simulink model "Der_Faux_FPGA_V2_optimized_synthesizable"  (R2020a)
settings: Solver=FixedStepDiscrete  StartTime=0.0  StopTime=0.84375  FixedStep=1/fs_sim  RelTol=1e-3
values from neighbouring files (symbols this model uses):
  ADC_res = 5    [Der_Faux_ctr_FPGA.m]
  ADC_res_G4 = 8    [Der_Faux_ctr_FPGA.m]
  fs = 48000    [Der_Faux_ctr_FPGA.m]
  fs_sim = fs*ovs    (= 6144000)    [Der_Faux_ctr_FPGA.m]
  Gvar1_N = fi(Gvar1_N,0,ADC_res,0)    [Der_Faux_ctr_FPGA.m]
  Gvar2_N = fi(Gvar2_N,0,ADC_res,0)    [Der_Faux_ctr_FPGA.m]
  Gvar3_N = fi(Gvar3_N,0,ADC_res,0)    [Der_Faux_ctr_FPGA.m]
  Gvar4_N = fi(Gvar4_N,0,ADC_res_G4,0)    [Der_Faux_ctr_FPGA.m]
  input_space = linspace(0,2^ADC_res-1,2^ADC_res)    [Der_Faux_ctr_FPGA.m]
  input_spcae_extended = linspace(0,(2^ADC_res)^3-1,(2^ADC_res)^3)    [Der_Faux_ctr_FPGA.m]
  LUT_Z22a_opt = sfi(LUT_Z22a, len_LUT22a)    [Der_Faux_ctr_FPGA.m]
  LUT_Z22b_opt = sfi(LUT_Z22b, len_LUT22b)    [Der_Faux_ctr_FPGA.m]
  LUT_Z23a_opt = sfi(LUT_Z23a, len_Z23a)    [Der_Faux_ctr_FPGA.m]
  LUT_Z23b_opt = sfi(LUT_Z23b, len_Z23b)    [Der_Faux_ctr_FPGA.m]
  LUT_Z24a_opt = sfi(LUT_Z24a, len_LUT24a)    [Der_Faux_ctr_FPGA.m]
  LUT_Z24b_opt = sfi(LUT_Z24b, len_LUT24b)    [Der_Faux_ctr_FPGA.m]
  LUT_Z25a_opt = sfi(LUT_Z25a, len_LUT25a)    [Der_Faux_ctr_FPGA.m]
  LUT_Z25b_opt = sfi(LUT_Z25b, len_LUT25b)    [Der_Faux_ctr_FPGA.m]
  shift_reg_size = 8*44000    (= 352000)    [Der_Faux_ctr_FPGA.m]
  use_stimuli = [true,true,true,true]    [Der_Faux_ctr_FPGA.m]
  WL_RAM = 5    [Der_Faux_ctr_FPGA.m]
undefined symbols (not defined in the file or in its folder): poti_stimuli1, poti_stimuli2, poti_stimuli3, poti_stimuli4
libraries: hdlmdlgenlib x30, simulink x6, hdlsllib x4
(part 2 of 3)

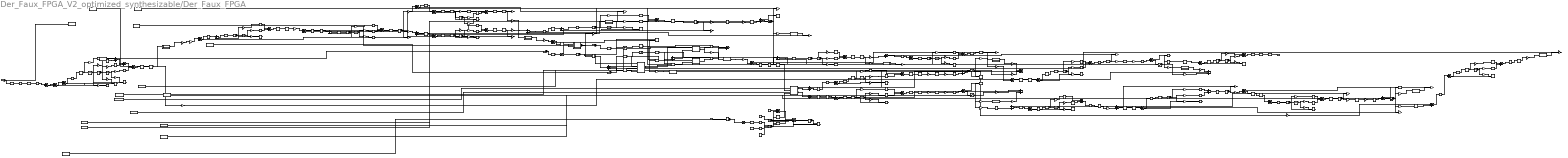
== system Der_Faux_FPGA_V2_optimized_synthesizable/Der_Faux_FPGA ==
  Vin : Inport  OutDataTypeStr=fixdt(1, 16, 15)  PortDimensions=1  SampleTime=2.08333333333333e-05  LockScale=on
  Gvar1_N : Inport  Port=2  OutDataTypeStr=fixdt(0, 5, 0)  PortDimensions=1  SampleTime=1.62760416666667e-07  LockScale=on
  Gvar2_N : Inport  Port=3  OutDataTypeStr=fixdt(0, 5, 0)  PortDimensions=1  SampleTime=1.62760416666667e-07  LockScale=on
  Gvar3_N : Inport  Port=4  OutDataTypeStr=fixdt(0, 5, 0)  PortDimensions=1  SampleTime=1.62760416666667e-07  LockScale=on
  Gvar4_N : Inport  Port=5  OutDataTypeStr=uint8  PortDimensions=1  SampleTime=1.62760416666667e-07  LockScale=on
  1-D Lookup Table1 : Lookup_n-D  NumberOfTableDimensions=1  BreakpointsForDimension1="fi(\"numerictype\",numerictype(0,8,0),\"fimath\",fimath(\"RoundingMethod\", \"Nearest\",\"OverflowAction\", \"Saturate\",\"ProductMode\",\"FullPrecision\",\"SumMode\",\"FullPrecision\"),\"Value\",\"[0 1 2 3 4 5 6 7 8 9 10 11 12 13 14 15 16 17 18 19 20 21 22 23 24 25 26 27 28 29 30 31 32 33 34 35 36 37 38 39 40 41 42 43 44 45 46 47 48 49 50 51 52 53 54 55 56 57 58 59 60 61 62 63 64 65 66 67 68 69 70 71 72 73 74 75 76 77 78 79 80 81 82 83 84 85 86 87 88 89 90 91 92 93 94 95 96 97 98 99 100 101 102 103 104 105 106 107 108 109 110 111 112 113 114 115 116 117 118 119 120 121 122 123 124 125 126 127 128 129 130 131 132 133 134 135 136 137 138 139 140 141 142 143 144 145 146 147 148 149 150 151 152 153 154 155 156 157 158 159 160 161 162 163 164 165 166 167 168 169 170 171 172 173 174 175 176 177 178 179 180 181 182 183 184 185 186 187 188 189 190 191 192 193 194 195 196 197 198 199 200 201 202 203 204 205 206 207 208 209 210 211 212 213 214 215 216 217 218 219 220 221 222 223 224 225 226 227 228 229 230 231 232 233 234 235 236 237 238 239 240 241 242 243 244 245 246 247 248 249 250 251 252 253 254 255]\")"  Table="reshape(fi(\"numerictype\",numerictype(0,4,0),\"fimath\",fimath(\"RoundingMethod\", \"Floor\",\"OverflowAction\", \"Wrap\",\"ProductMode\",\"FullPrecision\",\"SumMode\",\"FullPrecision\"),\"Value\",\"[1;1;1;1;1;1;1;1;1;1;1;1;1;1;1;1;1;1;1;1;1;1;1;1;1;1;1;1;1;1;1;1;1;1;1;1;1;1;1;1;1;1;1;1;1;1;1;1;1;1;1;2;2;2;2;2;2;2;2;2;2;2;2;2;2;2;2;2;2;2;2;2;2;2;2;2;3;3;3;3;3;3;3;3;3;3;3;3;3;3;3;3;3;3;3;3;3;3;3;3;3;3;4;4;4;4;4;4;4;4;4;4;4;4;4;4;4;4;4;4;4;4;4;4;4;4;4;5;5;5;5;5;5;5;5;5;5;5;5;5;5;5;5;5;5;5;5;5;5;5;5;5;5;6;6;6;6;6;6;6;6;6;6;6;6;6;6;6;6;6;6;6;6;6;6;6;6;6;7;7;7;7;7;7;7;7;7;7;7;7;7;7;7;7;7;7;7;7;7;7;7;7;7;7;8;8;8;8;8;8;8;8;8;8;8;8;8;8;8;8;8;8;8;8;8;8;8;8;8;9;9;9;9;9;9;9;9;9;9;9;9;9;9;9;9;9;9;9;9;9;9;9;9;9;9;10]\"), [1  256])"  InterpMethod=Flat  ExtrapMethod=Clip  DiagnosticForOutOfRangeInput=Error  SampleTime=1.62760416666667e-07  OutDataTypeStr=fixdt(0, 4, 0)  RndMeth=Simplest  InputSameDT=on
  Comparator Logic : Subsystem
  Compare To Zero2 : simulink/Logic and Bit Operations/Compare To Constant  relop===  const=double(0)  OutDataTypeStr=boolean
  Constant14 : Constant  Value=0  OutDataTypeStr=fixdt(0, 4, 0)  SampleTime=1.62760416666667e-07
  Constant8 : Constant  OutDataTypeStr=fixdt(0, 4, 0)  SampleTime=1.62760416666667e-07
  Data Type Conversion : DataTypeConversion  OutDataTypeStr=fixdt(1, 46, 44)  SampleTime=2.08333333333333e-05  SaturateOnIntegerOverflow=on
  Data Type Conversion1 : DataTypeConversion  OutDataTypeStr=fixdt(1, 16, 15)  SampleTime=2.08333333333333e-05  SaturateOnIntegerOverflow=on
  Data Type Conversion2 : DataTypeConversion  OutDataTypeStr=fixdt(0, 4, 0)  SampleTime=1.62760416666667e-07
  Delay Mod{1..6,8..9} (8 alike) : Delay  DelayLength=double(1)  InitialCondition=0  SampleTime=1.62760416666667e-07
  Delay1 : Delay  DelayLength=double(1)  InitialCondition=0  SampleTime=1.62760416666667e-07
  Delay2 : Delay  DelayLength=double(1)  InitialCondition=0  SampleTime=1.62760416666667e-07
  Delay3 : Delay  DelayLength=double(1)  InitialCondition=0  SampleTime=1.62760416666667e-07
  Difference1 : Subsystem  mask(Difference){ICPrevInput=double(0), InputProcessing=Elements as channels (sample based), OutMin=[], OutMax=[], OutDataTypeStr=fixdt(1,46,81), OutputDataTypeScalingMode=Specify via dialog, OutDataType=fixdt(1,46,81), OutScaling=[], LockScale=off, RndMeth=Floor, DoSatur=on}
      mask prompts: ICPrevInput "Simulink:masks:InitialConditionForPreviousInput_MP"; InputProcessing "Simulink:masks:InputProcessing_MP"; OutMin "Simulink:masks:OutputMinimum_MP"; OutMax "Simulink:masks:OutputMaximum_MP"; OutDataTypeStr "Simulink:masks:OutputDataType_MP"; OutputDataTypeScalingMode "Simulink:masks:OutputDataTypeMode_MP"; OutDataType "Simulink:masks:OutputDataTypeegFixdt116Fixdtsingle_MP"; OutScaling "Simulink:masks:OutputScalingSlopeEg29OrSlopeBias_MP"; LockScale "Simulink:masks:LockOutputDataTypeAgainstFxpTools_MP"; RndMeth "Simulink:masks:IntegerRoundingMode_MP"; DoSatur "Simulink:masks:SaturateToMaxOrMinWhenOverflowsOccur_MP"
      mask help: Simulink:masks:Difference_MD
      mask init:
      | blkH = gcbh;
      | blkName = getfullname(blkH);
      | 
      | set_param([blkName,'/Diff'], ...
      |     'RndMeth',RndMeth, ...
      | 	'DoSatur',DoSatur);
      | 
      | set_param([blkName,'/UD'], ...
      | 	'InputProcessing',InputProcessing);
      mask TypeOptions InputProcessing: Simulink:masks:ColumnsAsChannelsFrameBased | Simulink:masks:ElementsAsChannelsSampleBased
      mask Callback OutDataTypeStr: fixptdialog(gcbh)
      mask TypeOptions OutputDataTypeScalingMode: double | single | int8 | uint8 | int16 | uint16 | int32 | uint32 | Specify via dialog | Inherit via internal rule | Inherit via back propagation
      mask Callback OutputDataTypeScalingMode: fixptdialog(gcbh)
      mask Callback OutDataType: fixptdialog(gcbh)
      mask TypeOptions RndMeth: Simulink:masks:Ceiling | Simulink:masks:Convergent | Simulink:masks:Floor | Simulink:masks:Nearest | Simulink:masks:Round | Simulink:masks:Simplest | Simulink:masks:Zero
      mask Display: dpoly([1 -1],[1 0],'z')
  Difference10 : Subsystem  mask(Difference){ICPrevInput=double(0), InputProcessing=Elements as channels (sample based), OutMin=[], OutMax=[], OutDataTypeStr=fixdt(1,46,77), OutputDataTypeScalingMode=Specify via dialog, OutDataType=fixdt(1,46,77), OutScaling=[], LockScale=off, RndMeth=Floor, DoSatur=on}
      mask prompts: ICPrevInput "Simulink:masks:InitialConditionForPreviousInput_MP"; InputProcessing "Simulink:masks:InputProcessing_MP"; OutMin "Simulink:masks:OutputMinimum_MP"; OutMax "Simulink:masks:OutputMaximum_MP"; OutDataTypeStr "Simulink:masks:OutputDataType_MP"; OutputDataTypeScalingMode "Simulink:masks:OutputDataTypeMode_MP"; OutDataType "Simulink:masks:OutputDataTypeegFixdt116Fixdtsingle_MP"; OutScaling "Simulink:masks:OutputScalingSlopeEg29OrSlopeBias_MP"; LockScale "Simulink:masks:LockOutputDataTypeAgainstFxpTools_MP"; RndMeth "Simulink:masks:IntegerRoundingMode_MP"; DoSatur "Simulink:masks:SaturateToMaxOrMinWhenOverflowsOccur_MP"
      mask help: Simulink:masks:Difference_MD
      mask init:
      | blkH = gcbh;
      | blkName = getfullname(blkH);
      | 
      | set_param([blkName,'/Diff'], ...
      |     'RndMeth',RndMeth, ...
      | 	'DoSatur',DoSatur);
      | 
      | set_param([blkName,'/UD'], ...
      | 	'InputProcessing',InputProcessing);
      mask TypeOptions InputProcessing: Simulink:masks:ColumnsAsChannelsFrameBased | Simulink:masks:ElementsAsChannelsSampleBased
      mask Callback OutDataTypeStr: fixptdialog(gcbh)
      mask TypeOptions OutputDataTypeScalingMode: double | single | int8 | uint8 | int16 | uint16 | int32 | uint32 | Specify via dialog | Inherit via internal rule | Inherit via back propagation
      mask Callback OutputDataTypeScalingMode: fixptdialog(gcbh)
      mask Callback OutDataType: fixptdialog(gcbh)
      mask TypeOptions RndMeth: Simulink:masks:Ceiling | Simulink:masks:Convergent | Simulink:masks:Floor | Simulink:masks:Nearest | Simulink:masks:Round | Simulink:masks:Simplest | Simulink:masks:Zero
      mask Display: dpoly([1 -1],[1 0],'z')
  Difference11 : Subsystem  mask(Difference){ICPrevInput=double(0), InputProcessing=Elements as channels (sample based), OutMin=[], OutMax=[], OutDataTypeStr=fixdt(1,46,77), OutputDataTypeScalingMode=Specify via dialog, OutDataType=fixdt(1,46,77), OutScaling=[], LockScale=off, RndMeth=Floor, DoSatur=on}
      mask prompts: ICPrevInput "Simulink:masks:InitialConditionForPreviousInput_MP"; InputProcessing "Simulink:masks:InputProcessing_MP"; OutMin "Simulink:masks:OutputMinimum_MP"; OutMax "Simulink:masks:OutputMaximum_MP"; OutDataTypeStr "Simulink:masks:OutputDataType_MP"; OutputDataTypeScalingMode "Simulink:masks:OutputDataTypeMode_MP"; OutDataType "Simulink:masks:OutputDataTypeegFixdt116Fixdtsingle_MP"; OutScaling "Simulink:masks:OutputScalingSlopeEg29OrSlopeBias_MP"; LockScale "Simulink:masks:LockOutputDataTypeAgainstFxpTools_MP"; RndMeth "Simulink:masks:IntegerRoundingMode_MP"; DoSatur "Simulink:masks:SaturateToMaxOrMinWhenOverflowsOccur_MP"
      mask help: Simulink:masks:Difference_MD
      mask init:
      | blkH = gcbh;
      | blkName = getfullname(blkH);
      | 
      | set_param([blkName,'/Diff'], ...
      |     'RndMeth',RndMeth, ...
      | 	'DoSatur',DoSatur);
      | 
      | set_param([blkName,'/UD'], ...
      | 	'InputProcessing',InputProcessing);
      mask TypeOptions InputProcessing: Simulink:masks:ColumnsAsChannelsFrameBased | Simulink:masks:ElementsAsChannelsSampleBased
      mask Callback OutDataTypeStr: fixptdialog(gcbh)
      mask TypeOptions OutputDataTypeScalingMode: double | single | int8 | uint8 | int16 | uint16 | int32 | uint32 | Specify via dialog | Inherit via internal rule | Inherit via back propagation
      mask Callback OutputDataTypeScalingMode: fixptdialog(gcbh)
      mask Callback OutDataType: fixptdialog(gcbh)
      mask TypeOptions RndMeth: Simulink:masks:Ceiling | Simulink:masks:Convergent | Simulink:masks:Floor | Simulink:masks:Nearest | Simulink:masks:Round | Simulink:masks:Simplest | Simulink:masks:Zero
      mask Display: dpoly([1 -1],[1 0],'z')
  Difference12 : Subsystem  mask(Difference){ICPrevInput=double(0), InputProcessing=Elements as channels (sample based), OutMin=[], OutMax=[], OutDataTypeStr=fixdt(1,46,73), OutputDataTypeScalingMode=Specify via dialog, OutDataType=fixdt(1,46,73), OutScaling=[], LockScale=off, RndMeth=Floor, DoSatur=on}
      mask prompts: ICPrevInput "Simulink:masks:InitialConditionForPreviousInput_MP"; InputProcessing "Simulink:masks:InputProcessing_MP"; OutMin "Simulink:masks:OutputMinimum_MP"; OutMax "Simulink:masks:OutputMaximum_MP"; OutDataTypeStr "Simulink:masks:OutputDataType_MP"; OutputDataTypeScalingMode "Simulink:masks:OutputDataTypeMode_MP"; OutDataType "Simulink:masks:OutputDataTypeegFixdt116Fixdtsingle_MP"; OutScaling "Simulink:masks:OutputScalingSlopeEg29OrSlopeBias_MP"; LockScale "Simulink:masks:LockOutputDataTypeAgainstFxpTools_MP"; RndMeth "Simulink:masks:IntegerRoundingMode_MP"; DoSatur "Simulink:masks:SaturateToMaxOrMinWhenOverflowsOccur_MP"
      mask help: Simulink:masks:Difference_MD
      mask init:
      | blkH = gcbh;
      | blkName = getfullname(blkH);
      | 
      | set_param([blkName,'/Diff'], ...
      |     'RndMeth',RndMeth, ...
      | 	'DoSatur',DoSatur);
      | 
      | set_param([blkName,'/UD'], ...
      | 	'InputProcessing',InputProcessing);
      mask TypeOptions InputProcessing: Simulink:masks:ColumnsAsChannelsFrameBased | Simulink:masks:ElementsAsChannelsSampleBased
      mask Callback OutDataTypeStr: fixptdialog(gcbh)
      mask TypeOptions OutputDataTypeScalingMode: double | single | int8 | uint8 | int16 | uint16 | int32 | uint32 | Specify via dialog | Inherit via internal rule | Inherit via back propagation
      mask Callback OutputDataTypeScalingMode: fixptdialog(gcbh)
      mask Callback OutDataType: fixptdialog(gcbh)
      mask TypeOptions RndMeth: Simulink:masks:Ceiling | Simulink:masks:Convergent | Simulink:masks:Floor | Simulink:masks:Nearest | Simulink:masks:Round | Simulink:masks:Simplest | Simulink:masks:Zero
      mask Display: dpoly([1 -1],[1 0],'z')
  Difference13 : Subsystem  mask(Difference){ICPrevInput=double(0), InputProcessing=Elements as channels (sample based), OutMin=[], OutMax=[], OutDataTypeStr=fixdt(1,46,73), OutputDataTypeScalingMode=Specify via dialog, OutDataType=fixdt(1,46,73), OutScaling=[], LockScale=off, RndMeth=Floor, DoSatur=on}
      mask prompts: ICPrevInput "Simulink:masks:InitialConditionForPreviousInput_MP"; InputProcessing "Simulink:masks:InputProcessing_MP"; OutMin "Simulink:masks:OutputMinimum_MP"; OutMax "Simulink:masks:OutputMaximum_MP"; OutDataTypeStr "Simulink:masks:OutputDataType_MP"; OutputDataTypeScalingMode "Simulink:masks:OutputDataTypeMode_MP"; OutDataType "Simulink:masks:OutputDataTypeegFixdt116Fixdtsingle_MP"; OutScaling "Simulink:masks:OutputScalingSlopeEg29OrSlopeBias_MP"; LockScale "Simulink:masks:LockOutputDataTypeAgainstFxpTools_MP"; RndMeth "Simulink:masks:IntegerRoundingMode_MP"; DoSatur "Simulink:masks:SaturateToMaxOrMinWhenOverflowsOccur_MP"
      mask help: Simulink:masks:Difference_MD
      mask init:
      | blkH = gcbh;
      | blkName = getfullname(blkH);
      | 
      | set_param([blkName,'/Diff'], ...
      |     'RndMeth',RndMeth, ...
      | 	'DoSatur',DoSatur);
      | 
      | set_param([blkName,'/UD'], ...
      | 	'InputProcessing',InputProcessing);
      mask TypeOptions InputProcessing: Simulink:masks:ColumnsAsChannelsFrameBased | Simulink:masks:ElementsAsChannelsSampleBased
      mask Callback OutDataTypeStr: fixptdialog(gcbh)
      mask TypeOptions OutputDataTypeScalingMode: double | single | int8 | uint8 | int16 | uint16 | int32 | uint32 | Specify via dialog | Inherit via internal rule | Inherit via back propagation
      mask Callback OutputDataTypeScalingMode: fixptdialog(gcbh)
      mask Callback OutDataType: fixptdialog(gcbh)
      mask TypeOptions RndMeth: Simulink:masks:Ceiling | Simulink:masks:Convergent | Simulink:masks:Floor | Simulink:masks:Nearest | Simulink:masks:Round | Simulink:masks:Simplest | Simulink:masks:Zero
      mask Display: dpoly([1 -1],[1 0],'z')
  Difference3 : Subsystem  mask(Difference){ICPrevInput=double(0), InputProcessing=Elements as channels (sample based), OutMin=[], OutMax=[], OutDataTypeStr=fixdt(1,46,47), OutputDataTypeScalingMode=Specify via dialog, OutDataType=fixdt(1,46,47), OutScaling=[], LockScale=off, RndMeth=Floor, DoSatur=on}
      mask prompts: ICPrevInput "Simulink:masks:InitialConditionForPreviousInput_MP"; InputProcessing "Simulink:masks:InputProcessing_MP"; OutMin "Simulink:masks:OutputMinimum_MP"; OutMax "Simulink:masks:OutputMaximum_MP"; OutDataTypeStr "Simulink:masks:OutputDataType_MP"; OutputDataTypeScalingMode "Simulink:masks:OutputDataTypeMode_MP"; OutDataType "Simulink:masks:OutputDataTypeegFixdt116Fixdtsingle_MP"; OutScaling "Simulink:masks:OutputScalingSlopeEg29OrSlopeBias_MP"; LockScale "Simulink:masks:LockOutputDataTypeAgainstFxpTools_MP"; RndMeth "Simulink:masks:IntegerRoundingMode_MP"; DoSatur "Simulink:masks:SaturateToMaxOrMinWhenOverflowsOccur_MP"
      mask help: Simulink:masks:Difference_MD
      mask init:
      | blkH = gcbh;
      | blkName = getfullname(blkH);
      | 
      | set_param([blkName,'/Diff'], ...
      |     'RndMeth',RndMeth, ...
      | 	'DoSatur',DoSatur);
      | 
      | set_param([blkName,'/UD'], ...
      | 	'InputProcessing',InputProcessing);
      mask TypeOptions InputProcessing: Simulink:masks:ColumnsAsChannelsFrameBased | Simulink:masks:ElementsAsChannelsSampleBased
      mask Callback OutDataTypeStr: fixptdialog(gcbh)
      mask TypeOptions OutputDataTypeScalingMode: double | single | int8 | uint8 | int16 | uint16 | int32 | uint32 | Specify via dialog | Inherit via internal rule | Inherit via back propagation
      mask Callback OutputDataTypeScalingMode: fixptdialog(gcbh)
      mask Callback OutDataType: fixptdialog(gcbh)
      mask TypeOptions RndMeth: Simulink:masks:Ceiling | Simulink:masks:Convergent | Simulink:masks:Floor | Simulink:masks:Nearest | Simulink:masks:Round | Simulink:masks:Simplest | Simulink:masks:Zero
      mask Display: dpoly([1 -1],[1 0],'z')
  Difference4 : Subsystem  mask(Difference){ICPrevInput=double(0), InputProcessing=Elements as channels (sample based), OutMin=[], OutMax=[], OutDataTypeStr=fixdt(1,46,82), OutputDataTypeScalingMode=Specify via dialog, OutDataType=fixdt(1,46,82), OutScaling=[], LockScale=off, RndMeth=Floor, DoSatur=on}
      mask prompts: ICPrevInput "Simulink:masks:InitialConditionForPreviousInput_MP"; InputProcessing "Simulink:masks:InputProcessing_MP"; OutMin "Simulink:masks:OutputMinimum_MP"; OutMax "Simulink:masks:OutputMaximum_MP"; OutDataTypeStr "Simulink:masks:OutputDataType_MP"; OutputDataTypeScalingMode "Simulink:masks:OutputDataTypeMode_MP"; OutDataType "Simulink:masks:OutputDataTypeegFixdt116Fixdtsingle_MP"; OutScaling "Simulink:masks:OutputScalingSlopeEg29OrSlopeBias_MP"; LockScale "Simulink:masks:LockOutputDataTypeAgainstFxpTools_MP"; RndMeth "Simulink:masks:IntegerRoundingMode_MP"; DoSatur "Simulink:masks:SaturateToMaxOrMinWhenOverflowsOccur_MP"
      mask help: Simulink:masks:Difference_MD
      mask init:
      | blkH = gcbh;
      | blkName = getfullname(blkH);
      | 
      | set_param([blkName,'/Diff'], ...
      |     'RndMeth',RndMeth, ...
      | 	'DoSatur',DoSatur);
      | 
      | set_param([blkName,'/UD'], ...
      | 	'InputProcessing',InputProcessing);
      mask TypeOptions InputProcessing: Simulink:masks:ColumnsAsChannelsFrameBased | Simulink:masks:ElementsAsChannelsSampleBased
      mask Callback OutDataTypeStr: fixptdialog(gcbh)
      mask TypeOptions OutputDataTypeScalingMode: double | single | int8 | uint8 | int16 | uint16 | int32 | uint32 | Specify via dialog | Inherit via internal rule | Inherit via back propagation
      mask Callback OutputDataTypeScalingMode: fixptdialog(gcbh)
      mask Callback OutDataType: fixptdialog(gcbh)
      mask TypeOptions RndMeth: Simulink:masks:Ceiling | Simulink:masks:Convergent | Simulink:masks:Floor | Simulink:masks:Nearest | Simulink:masks:Round | Simulink:masks:Simplest | Simulink:masks:Zero
      mask Display: dpoly([1 -1],[1 0],'z')
  Difference5 : Subsystem  mask(Difference){ICPrevInput=double(0), InputProcessing=Elements as channels (sample based), OutMin=[], OutMax=[], OutDataTypeStr=fixdt(1,46,76), OutputDataTypeScalingMode=Specify via dialog, OutDataType=fixdt(1,46,76), OutScaling=[], LockScale=off, RndMeth=Floor, DoSatur=on}
      mask prompts: ICPrevInput "Simulink:masks:InitialConditionForPreviousInput_MP"; InputProcessing "Simulink:masks:InputProcessing_MP"; OutMin "Simulink:masks:OutputMinimum_MP"; OutMax "Simulink:masks:OutputMaximum_MP"; OutDataTypeStr "Simulink:masks:OutputDataType_MP"; OutputDataTypeScalingMode "Simulink:masks:OutputDataTypeMode_MP"; OutDataType "Simulink:masks:OutputDataTypeegFixdt116Fixdtsingle_MP"; OutScaling "Simulink:masks:OutputScalingSlopeEg29OrSlopeBias_MP"; LockScale "Simulink:masks:LockOutputDataTypeAgainstFxpTools_MP"; RndMeth "Simulink:masks:IntegerRoundingMode_MP"; DoSatur "Simulink:masks:SaturateToMaxOrMinWhenOverflowsOccur_MP"
      mask help: Simulink:masks:Difference_MD
      mask init:
      | blkH = gcbh;
      | blkName = getfullname(blkH);
      | 
      | set_param([blkName,'/Diff'], ...
      |     'RndMeth',RndMeth, ...
      | 	'DoSatur',DoSatur);
      | 
      | set_param([blkName,'/UD'], ...
      | 	'InputProcessing',InputProcessing);
      mask TypeOptions InputProcessing: Simulink:masks:ColumnsAsChannelsFrameBased | Simulink:masks:ElementsAsChannelsSampleBased
      mask Callback OutDataTypeStr: fixptdialog(gcbh)
      mask TypeOptions OutputDataTypeScalingMode: double | single | int8 | uint8 | int16 | uint16 | int32 | uint32 | Specify via dialog | Inherit via internal rule | Inherit via back propagation
      mask Callback OutputDataTypeScalingMode: fixptdialog(gcbh)
      mask Callback OutDataType: fixptdialog(gcbh)
      mask TypeOptions RndMeth: Simulink:masks:Ceiling | Simulink:masks:Convergent | Simulink:masks:Floor | Simulink:masks:Nearest | Simulink:masks:Round | Simulink:masks:Simplest | Simulink:masks:Zero
      mask Display: dpoly([1 -1],[1 0],'z')
  Difference6 : Subsystem  mask(Difference){ICPrevInput=double(0), InputProcessing=Elements as channels (sample based), OutMin=[], OutMax=[], OutDataTypeStr=fixdt(1,46,76), OutputDataTypeScalingMode=Specify via dialog, OutDataType=fixdt(1,46,76), OutScaling=[], LockScale=off, RndMeth=Floor, DoSatur=on}
      mask prompts: ICPrevInput "Simulink:masks:InitialConditionForPreviousInput_MP"; InputProcessing "Simulink:masks:InputProcessing_MP"; OutMin "Simulink:masks:OutputMinimum_MP"; OutMax "Simulink:masks:OutputMaximum_MP"; OutDataTypeStr "Simulink:masks:OutputDataType_MP"; OutputDataTypeScalingMode "Simulink:masks:OutputDataTypeMode_MP"; OutDataType "Simulink:masks:OutputDataTypeegFixdt116Fixdtsingle_MP"; OutScaling "Simulink:masks:OutputScalingSlopeEg29OrSlopeBias_MP"; LockScale "Simulink:masks:LockOutputDataTypeAgainstFxpTools_MP"; RndMeth "Simulink:masks:IntegerRoundingMode_MP"; DoSatur "Simulink:masks:SaturateToMaxOrMinWhenOverflowsOccur_MP"
      mask help: Simulink:masks:Difference_MD
      mask init:
      | blkH = gcbh;
      | blkName = getfullname(blkH);
      | 
      | set_param([blkName,'/Diff'], ...
      |     'RndMeth',RndMeth, ...
      | 	'DoSatur',DoSatur);
      | 
      | set_param([blkName,'/UD'], ...
      | 	'InputProcessing',InputProcessing);
      mask TypeOptions InputProcessing: Simulink:masks:ColumnsAsChannelsFrameBased | Simulink:masks:ElementsAsChannelsSampleBased
      mask Callback OutDataTypeStr: fixptdialog(gcbh)
      mask TypeOptions OutputDataTypeScalingMode: double | single | int8 | uint8 | int16 | uint16 | int32 | uint32 | Specify via dialog | Inherit via internal rule | Inherit via back propagation
      mask Callback OutputDataTypeScalingMode: fixptdialog(gcbh)
      mask Callback OutDataType: fixptdialog(gcbh)
      mask TypeOptions RndMeth: Simulink:masks:Ceiling | Simulink:masks:Convergent | Simulink:masks:Floor | Simulink:masks:Nearest | Simulink:masks:Round | Simulink:masks:Simplest | Simulink:masks:Zero
      mask Display: dpoly([1 -1],[1 0],'z')
  Difference7 : Subsystem  mask(Difference){ICPrevInput=double(0), InputProcessing=Elements as channels (sample based), OutMin=[], OutMax=[], OutDataTypeStr=fixdt(1,46,83), OutputDataTypeScalingMode=Specify via dialog, OutDataType=fixdt(1,46,83), OutScaling=[], LockScale=off, RndMeth=Floor, DoSatur=on}
      mask prompts: ICPrevInput "Simulink:masks:InitialConditionForPreviousInput_MP"; InputProcessing "Simulink:masks:InputProcessing_MP"; OutMin "Simulink:masks:OutputMinimum_MP"; OutMax "Simulink:masks:OutputMaximum_MP"; OutDataTypeStr "Simulink:masks:OutputDataType_MP"; OutputDataTypeScalingMode "Simulink:masks:OutputDataTypeMode_MP"; OutDataType "Simulink:masks:OutputDataTypeegFixdt116Fixdtsingle_MP"; OutScaling "Simulink:masks:OutputScalingSlopeEg29OrSlopeBias_MP"; LockScale "Simulink:masks:LockOutputDataTypeAgainstFxpTools_MP"; RndMeth "Simulink:masks:IntegerRoundingMode_MP"; DoSatur "Simulink:masks:SaturateToMaxOrMinWhenOverflowsOccur_MP"
      mask help: Simulink:masks:Difference_MD
      mask init:
      | blkH = gcbh;
      | blkName = getfullname(blkH);
      | 
      | set_param([blkName,'/Diff'], ...
      |     'RndMeth',RndMeth, ...
      | 	'DoSatur',DoSatur);
      | 
      | set_param([blkName,'/UD'], ...
      | 	'InputProcessing',InputProcessing);
      mask TypeOptions InputProcessing: Simulink:masks:ColumnsAsChannelsFrameBased | Simulink:masks:ElementsAsChannelsSampleBased
      mask Callback OutDataTypeStr: fixptdialog(gcbh)
      mask TypeOptions OutputDataTypeScalingMode: double | single | int8 | uint8 | int16 | uint16 | int32 | uint32 | Specify via dialog | Inherit via internal rule | Inherit via back propagation
      mask Callback OutputDataTypeScalingMode: fixptdialog(gcbh)
      mask Callback OutDataType: fixptdialog(gcbh)
      mask TypeOptions RndMeth: Simulink:masks:Ceiling | Simulink:masks:Convergent | Simulink:masks:Floor | Simulink:masks:Nearest | Simulink:masks:Round | Simulink:masks:Simplest | Simulink:masks:Zero
      mask Display: dpoly([1 -1],[1 0],'z')
  Difference8 : Subsystem  mask(Difference){ICPrevInput=double(0), InputProcessing=Elements as channels (sample based), OutMin=[], OutMax=[], OutDataTypeStr=fixdt(1,46,73), OutputDataTypeScalingMode=Specify via dialog, OutDataType=fixdt(1,46,73), OutScaling=[], LockScale=off, RndMeth=Floor, DoSatur=on}
      mask prompts: ICPrevInput "Simulink:masks:InitialConditionForPreviousInput_MP"; InputProcessing "Simulink:masks:InputProcessing_MP"; OutMin "Simulink:masks:OutputMinimum_MP"; OutMax "Simulink:masks:OutputMaximum_MP"; OutDataTypeStr "Simulink:masks:OutputDataType_MP"; OutputDataTypeScalingMode "Simulink:masks:OutputDataTypeMode_MP"; OutDataType "Simulink:masks:OutputDataTypeegFixdt116Fixdtsingle_MP"; OutScaling "Simulink:masks:OutputScalingSlopeEg29OrSlopeBias_MP"; LockScale "Simulink:masks:LockOutputDataTypeAgainstFxpTools_MP"; RndMeth "Simulink:masks:IntegerRoundingMode_MP"; DoSatur "Simulink:masks:SaturateToMaxOrMinWhenOverflowsOccur_MP"
      mask help: Simulink:masks:Difference_MD
      mask init:
      | blkH = gcbh;
      | blkName = getfullname(blkH);
      | 
      | set_param([blkName,'/Diff'], ...
      |     'RndMeth',RndMeth, ...
      | 	'DoSatur',DoSatur);
      | 
      | set_param([blkName,'/UD'], ...
      | 	'InputProcessing',InputProcessing);
      mask TypeOptions InputProcessing: Simulink:masks:ColumnsAsChannelsFrameBased | Simulink:masks:ElementsAsChannelsSampleBased
      mask Callback OutDataTypeStr: fixptdialog(gcbh)
      mask TypeOptions OutputDataTypeScalingMode: double | single | int8 | uint8 | int16 | uint16 | int32 | uint32 | Specify via dialog | Inherit via internal rule | Inherit via back propagation
      mask Callback OutputDataTypeScalingMode: fixptdialog(gcbh)
      mask Callback OutDataType: fixptdialog(gcbh)
      mask TypeOptions RndMeth: Simulink:masks:Ceiling | Simulink:masks:Convergent | Simulink:masks:Floor | Simulink:masks:Nearest | Simulink:masks:Round | Simulink:masks:Simplest | Simulink:masks:Zero
      mask Display: dpoly([1 -1],[1 0],'z')
  Difference9 : Subsystem  mask(Difference){ICPrevInput=double(0), InputProcessing=Elements as channels (sample based), OutMin=[], OutMax=[], OutDataTypeStr=fixdt(1,46,73), OutputDataTypeScalingMode=Specify via dialog, OutDataType=fixdt(1,46,73), OutScaling=[], LockScale=off, RndMeth=Floor, DoSatur=on}
      mask prompts: ICPrevInput "Simulink:masks:InitialConditionForPreviousInput_MP"; InputProcessing "Simulink:masks:InputProcessing_MP"; OutMin "Simulink:masks:OutputMinimum_MP"; OutMax "Simulink:masks:OutputMaximum_MP"; OutDataTypeStr "Simulink:masks:OutputDataType_MP"; OutputDataTypeScalingMode "Simulink:masks:OutputDataTypeMode_MP"; OutDataType "Simulink:masks:OutputDataTypeegFixdt116Fixdtsingle_MP"; OutScaling "Simulink:masks:OutputScalingSlopeEg29OrSlopeBias_MP"; LockScale "Simulink:masks:LockOutputDataTypeAgainstFxpTools_MP"; RndMeth "Simulink:masks:IntegerRoundingMode_MP"; DoSatur "Simulink:masks:SaturateToMaxOrMinWhenOverflowsOccur_MP"
      mask help: Simulink:masks:Difference_MD
      mask init:
      | blkH = gcbh;
      | blkName = getfullname(blkH);
      | 
      | set_param([blkName,'/Diff'], ...
      |     'RndMeth',RndMeth, ...
      | 	'DoSatur',DoSatur);
      | 
      | set_param([blkName,'/UD'], ...
      | 	'InputProcessing',InputProcessing);
      mask TypeOptions InputProcessing: Simulink:masks:ColumnsAsChannelsFrameBased | Simulink:masks:ElementsAsChannelsSampleBased
      mask Callback OutDataTypeStr: fixptdialog(gcbh)
      mask TypeOptions OutputDataTypeScalingMode: double | single | int8 | uint8 | int16 | uint16 | int32 | uint32 | Specify via dialog | Inherit via internal rule | Inherit via back propagation
      mask Callback OutputDataTypeScalingMode: fixptdialog(gcbh)
      mask Callback OutDataType: fixptdialog(gcbh)
      mask TypeOptions RndMeth: Simulink:masks:Ceiling | Simulink:masks:Convergent | Simulink:masks:Floor | Simulink:masks:Nearest | Simulink:masks:Round | Simulink:masks:Simplest | Simulink:masks:Zero
      mask Display: dpoly([1 -1],[1 0],'z')
  Discrete-Time Integrator1_reg : Delay  DelayLength=double(1)  InitialCondition=0  SampleTime=1.62760416666667e-07
  Discrete-Time Integrator1_saturate : Saturate  UpperLimit="fi(0,1,46,43,\"hex\",\"140000000000\")"  LowerLimit="fi(0,1,46,43,\"hex\",\"2c0000000000\")"  SampleTime=1.62760416666667e-07  OutDataTypeStr=fixdt(1, 46, 43)
  Discrete-Time Integrator2_reg : Delay  DelayLength=double(1)  InitialCondition=0  SampleTime=1.62760416666667e-07
  Discrete-Time Integrator2_saturate : Saturate  UpperLimit="fi(0,1,46,42,\"hex\",\"120000000000\")"  LowerLimit="fi(0,1,46,42,\"hex\",\"2e0000000000\")"  SampleTime=1.62760416666667e-07  OutDataTypeStr=fixdt(1, 46, 42)
  Discrete-Time Integrator4_reg : Delay  DelayLength=double(1)  InitialCondition=0  SampleTime=1.62760416666667e-07
  Discrete-Time Integrator4_saturate : Saturate  UpperLimit="fi(0,1,46,42,\"hex\",\"0a0000000000\")"  LowerLimit="fi(0,1,46,42,\"hex\",\"360000000000\")"  SampleTime=1.62760416666667e-07  OutDataTypeStr=fixdt(1, 46, 42)
  Discrete-Time Integrator5_reg : Delay  DelayLength=double(1)  InitialCondition=0  SampleTime=1.62760416666667e-07
  Discrete-Time Integrator5_saturate : Saturate  UpperLimit="fi(0,1,46,42,\"hex\",\"0a0000000000\")"  LowerLimit="fi(0,1,46,42,\"hex\",\"360000000000\")"  SampleTime=1.62760416666667e-07  OutDataTypeStr=fixdt(1, 46, 42)
  Discrete-Time Integrator6_reg : Delay  DelayLength=double(1)  InitialCondition=0  SampleTime=1.62760416666667e-07
  Discrete-Time Integrator6_saturate : Saturate  UpperLimit="fi(0,1,46,42,\"hex\",\"0a0000000000\")"  LowerLimit="fi(0,1,46,42,\"hex\",\"360000000000\")"  SampleTime=1.62760416666667e-07  OutDataTypeStr=fixdt(1, 46, 42)
  Gain10 : Gain  Gain="fi(0,1,46,22,\"hex\",\"177000000000\")"  ParamDataTypeStr=fixdt(1, 46, 22)  OutDataTypeStr=fixdt(1, 46, 59)  SaturateOnIntegerOverflow=on  SampleTime=1.62760416666667e-07
  Gain{12,14,16,59} (4 alike) : Gain  Gain="fi(0,1,46,58,\"hex\",\"15d867c3ece3\")"  ParamDataTypeStr=fixdt(1, 46, 58)  OutDataTypeStr=fixdt(1, 46, 56)  SaturateOnIntegerOverflow=on  SampleTime=1.62760416666667e-07
  Gain13 : Gain  Gain="fi(0,1,46,22,\"hex\",\"177000000000\")"  ParamDataTypeStr=fixdt(1, 46, 22)  OutDataTypeStr=fixdt(1, 46, 25)  SaturateOnIntegerOverflow=on  SampleTime=1.62760416666667e-07
  Gain{8,15,17..18,47} (5 alike) : Gain  Gain="fi(0,1,46,58,\"hex\",\"15d867c3ece3\")"  ParamDataTypeStr=fixdt(1, 46, 58)  OutDataTypeStr=fixdt(1, 46, 57)  SaturateOnIntegerOverflow=on  SampleTime=1.62760416666667e-07
  Gain19 : Gain  Gain="fi(0,1,46,25,\"hex\",\"217b80000000\")"  ParamDataTypeStr=fixdt(1, 46, 25)  OutDataTypeStr=fixdt(1, 46, 24)  SaturateOnIntegerOverflow=on  SampleTime=1.62760416666667e-07
  Gain20 : Gain  Gain="fi(0,1,46,75,\"hex\",\"175d57df90fb\")"  ParamDataTypeStr=fixdt(1, 46, 75)  OutDataTypeStr=fixdt(1, 46, 73)  SaturateOnIntegerOverflow=on  SampleTime=1.62760416666667e-07
  Gain23 : Gain  Gain="fi(0,1,46,58,\"hex\",\"1a36e2eb1c43\")"  ParamDataTypeStr=fixdt(1, 46, 58)  OutDataTypeStr=fixdt(1, 46, 63)  SaturateOnIntegerOverflow=on  SampleTime=1.62760416666667e-07
  Gain24 : Gain  Gain="fi(0,1,46,58,\"hex\",\"1a36e2eb1c43\")"  ParamDataTypeStr=fixdt(1, 46, 58)  OutDataTypeStr=fixdt(1, 46, 57)  SaturateOnIntegerOverflow=on  SampleTime=1.62760416666667e-07
  Gain25 : Gain  Gain="fi(0,1,46,58,\"hex\",\"1a36e2eb1c43\")"  ParamDataTypeStr=fixdt(1, 46, 58)  OutDataTypeStr=fixdt(1, 46, 57)  SaturateOnIntegerOverflow=on  SampleTime=1.62760416666667e-07
  Gain26 : Gain  Gain="fi(0,1,46,58,\"hex\",\"1a36e2eb1c43\")"  ParamDataTypeStr=fixdt(1, 46, 58)  OutDataTypeStr=fixdt(1, 46, 56)  SaturateOnIntegerOverflow=on  SampleTime=1.62760416666667e-07
  Gain27 : Gain  Gain="fi(0,1,46,64,\"hex\",\"10c6f7a0b5ee\")"  ParamDataTypeStr=fixdt(1, 46, 64)  OutDataTypeStr=fixdt(1, 46, 63)  SaturateOnIntegerOverflow=on  SampleTime=1.62760416666667e-07
  Gain28 : Gain  Gain="fi(0,1,46,64,\"hex\",\"10c6f7a0b5ee\")"  ParamDataTypeStr=fixdt(1, 46, 64)  OutDataTypeStr=fixdt(1, 46, 62)  SaturateOnIntegerOverflow=on  SampleTime=1.62760416666667e-07
  Gain29 : Gain  Gain="fi(0,1,46,68,\"hex\",\"1ad7f29abcaf\")"  ParamDataTypeStr=fixdt(1, 46, 68)  OutDataTypeStr=fixdt(1, 46, 66)  SaturateOnIntegerOverflow=on  SampleTime=1.62760416666667e-07
  Gain30 : Gain  Gain="fi(0,1,46,68,\"hex\",\"1ad7f29abcaf\")"  ParamDataTypeStr=fixdt(1, 46, 68)  OutDataTypeStr=fixdt(1, 46, 66)  SaturateOnIntegerOverflow=on  SampleTime=1.62760416666667e-07
  Gain31 : Gain  Gain="fi(0,1,46,59,\"hex\",\"1a36e2eb1c43\")"  ParamDataTypeStr=fixdt(1, 46, 59)  OutDataTypeStr=fixdt(1, 46, 57)  SaturateOnIntegerOverflow=on  SampleTime=1.62760416666667e-07
  Gain32 : Gain  Gain="fi(0,1,46,59,\"hex\",\"1a36e2eb1c43\")"  ParamDataTypeStr=fixdt(1, 46, 59)  OutDataTypeStr=fixdt(1, 46, 57)  SaturateOnIntegerOverflow=on  SampleTime=1.62760416666667e-07
  Gain33 : Gain  Gain="fi(0,1,46,64,\"hex\",\"10c6f7a0b5ee\")"  ParamDataTypeStr=fixdt(1, 46, 64)  OutDataTypeStr=fixdt(1, 46, 63)  SaturateOnIntegerOverflow=on  SampleTime=1.62760416666667e-07
  Gain34 : Gain  Gain="fi(0,1,46,64,\"hex\",\"10c6f7a0b5ee\")"  ParamDataTypeStr=fixdt(1, 46, 64)  OutDataTypeStr=fixdt(1, 46, 62)  SaturateOnIntegerOverflow=on  SampleTime=1.62760416666667e-07
  Gain42 : Gain  Gain="fi(0,1,46,22,\"hex\",\"177000000000\")"  ParamDataTypeStr=fixdt(1, 46, 22)  OutDataTypeStr=fixdt(1, 46, 59)  SaturateOnIntegerOverflow=on  SampleTime=1.62760416666667e-07
  Gain43 : Gain  Gain="fi(0,1,46,58,\"hex\",\"15d867c3ece3\")"  ParamDataTypeStr=fixdt(1, 46, 58)  OutDataTypeStr=fixdt(1, 46, 60)  SaturateOnIntegerOverflow=on  SampleTime=1.62760416666667e-07
  Gain44 : Gain  Gain="fi(0,1,46,22,\"hex\",\"177000000000\")"  ParamDataTypeStr=fixdt(1, 46, 22)  OutDataTypeStr=fixdt(1, 46, 53)  SaturateOnIntegerOverflow=on  SampleTime=1.62760416666667e-07
  Gain45 : Gain  Gain="fi(0,1,46,22,\"hex\",\"177000000000\")"  ParamDataTypeStr=fixdt(1, 46, 22)  OutDataTypeStr=fixdt(1, 46, 53)  SaturateOnIntegerOverflow=on  SampleTime=1.62760416666667e-07
  Gain46 : Gain  Gain="fi(0,1,46,22,\"hex\",\"177000000000\")"  ParamDataTypeStr=fixdt(1, 46, 22)  OutDataTypeStr=fixdt(1, 46, 60)  SaturateOnIntegerOverflow=on  SampleTime=1.62760416666667e-07
  Gain48 : Gain  Gain="fi(0,1,46,58,\"hex\",\"15d867c3ece3\")"  ParamDataTypeStr=fixdt(1, 46, 58)  OutDataTypeStr=fixdt(1, 46, 60)  SaturateOnIntegerOverflow=on  SampleTime=1.62760416666667e-07
  Gain49 : Gain  Gain="fi(0,1,46,58,\"hex\",\"15d867c3ece3\")"  ParamDataTypeStr=fixdt(1, 46, 58)  OutDataTypeStr=fixdt(1, 46, 64)  SaturateOnIntegerOverflow=on  SampleTime=1.62760416666667e-07
  Gain5 : Gain  Gain="fi(0,1,46,59,\"hex\",\"17d4ce4a19b1\")"  ParamDataTypeStr=fixdt(1, 46, 59)  OutDataTypeStr=fixdt(1, 46, 57)  SaturateOnIntegerOverflow=on  SampleTime=1.62760416666667e-07
  Gain50 : Gain  Gain="fi(0,1,46,59,\"hex\",\"17d4ce4a19b1\")"  ParamDataTypeStr=fixdt(1, 46, 59)  OutDataTypeStr=fixdt(1, 46, 57)  SaturateOnIntegerOverflow=on  SampleTime=1.62760416666667e-07
  Gain51 : Gain  Gain="fi(0,1,46,25,\"hex\",\"217b80000000\")"  ParamDataTypeStr=fixdt(1, 46, 25)  OutDataTypeStr=fixdt(1, 46, 23)  SaturateOnIntegerOverflow=on  SampleTime=1.62760416666667e-07
  Gain52 : Gain  Gain="fi(0,1,46,25,\"hex\",\"217b80000000\")"  ParamDataTypeStr=fixdt(1, 46, 25)  OutDataTypeStr=fixdt(1, 46, 23)  SaturateOnIntegerOverflow=on  SampleTime=1.62760416666667e-07
  Gain53 : Gain  Gain="fi(0,1,46,57,\"hex\",\"1be33da86a52\")"  ParamDataTypeStr=fixdt(1, 46, 57)  OutDataTypeStr=fixdt(1, 46, 55)  SaturateOnIntegerOverflow=on  SampleTime=1.62760416666667e-07
  Gain54 : Gain  Gain="fi(0,1,46,68,\"hex\",\"1240eca6a944\")"  ParamDataTypeStr=fixdt(1, 46, 68)  OutDataTypeStr=fixdt(1, 46, 66)  SaturateOnIntegerOverflow=on  SampleTime=1.62760416666667e-07
  Gain55 : Gain  Gain="fi(0,1,46,57,\"hex\",\"1be33da86a52\")"  ParamDataTypeStr=fixdt(1, 46, 57)  OutDataTypeStr=fixdt(1, 46, 55)  SaturateOnIntegerOverflow=on  SampleTime=1.62760416666667e-07
  Gain56 : Gain  Gain="fi(0,1,46,67,\"hex\",\"1421f5f40d83\")"  ParamDataTypeStr=fixdt(1, 46, 67)  OutDataTypeStr=fixdt(1, 46, 65)  SaturateOnIntegerOverflow=on  SampleTime=1.62760416666667e-07
  Gain57 : Gain  Gain="fi(0,1,46,22,\"hex\",\"177000000000\")"  ParamDataTypeStr=fixdt(1, 46, 22)  OutDataTypeStr=fixdt(1, 46, 50)  SaturateOnIntegerOverflow=on  SampleTime=1.62760416666667e-07
  Gain6 : Gain  Gain="fi(0,1,46,64,\"hex\",\"10c6f7a0b5ee\")"  ParamDataTypeStr=fixdt(1, 46, 64)  OutDataTypeStr=fixdt(1, 46, 45)  SaturateOnIntegerOverflow=on  SampleTime=1.62760416666667e-07
  Gain60 : Gain  Gain="fi(0,1,46,60,\"hex\",\"164f6486bb75\")"  ParamDataTypeStr=fixdt(1, 46, 60)  OutDataTypeStr=fixdt(1, 46, 58)  SaturateOnIntegerOverflow=on  SampleTime=1.62760416666667e-07
  Gain61 : Gain  Gain="fi(0,1,46,25,\"hex\",\"217b80000000\")"  ParamDataTypeStr=fixdt(1, 46, 25)  OutDataTypeStr=fixdt(1, 46, 30)  SaturateOnIntegerOverflow=on  SampleTime=1.62760416666667e-07
  Gain62 : Gain  Gain="fi(0,1,46,56,\"hex\",\"1845c8a0ce51\")"  ParamDataTypeStr=fixdt(1, 46, 56)  OutDataTypeStr=fixdt(1, 46, 54)  SaturateOnIntegerOverflow=on  SampleTime=1.62760416666667e-07
  Gain63 : Gain  Gain="fi(0,1,46,74,\"hex\",\"112e0be826d7\")"  ParamDataTypeStr=fixdt(1, 46, 74)  OutDataTypeStr=fixdt(1, 46, 73)  SaturateOnIntegerOverflow=on  SampleTime=1.62760416666667e-07
  Gain64 : Gain  Gain="fi(0,1,46,22,\"hex\",\"177000000000\")"  ParamDataTypeStr=fixdt(1, 46, 22)  OutDataTypeStr=fixdt(1, 46, 50)  SaturateOnIntegerOverflow=on  SampleTime=1.62760416666667e-07
  Gain65 : Gain  Gain="fi(0,1,46,22,\"hex\",\"177000000000\")"  ParamDataTypeStr=fixdt(1, 46, 22)  OutDataTypeStr=fixdt(1, 46, 54)  SaturateOnIntegerOverflow=on  SampleTime=1.62760416666667e-07
  Gain66 : Gain  Gain="fi(0,1,46,22,\"hex\",\"177000000000\")"  ParamDataTypeStr=fixdt(1, 46, 22)  OutDataTypeStr=fixdt(1, 46, 54)  SaturateOnIntegerOverflow=on  SampleTime=1.62760416666667e-07
  Gain67 : Gain  Gain="fi(0,1,46,22,\"hex\",\"177000000000\")"  ParamDataTypeStr=fixdt(1, 46, 22)  OutDataTypeStr=fixdt(1, 46, 51)  SaturateOnIntegerOverflow=on  SampleTime=1.62760416666667e-07
  Gain68 : Gain  Gain="fi(0,1,46,22,\"hex\",\"177000000000\")"  ParamDataTypeStr=fixdt(1, 46, 22)  OutDataTypeStr=fixdt(1, 46, 51)  SaturateOnIntegerOverflow=on  SampleTime=1.62760416666667e-07
  Gain7 : Gain  Gain="fi(0,1,46,20,\"hex\",\"2e060ec14161\")"  ParamDataTypeStr=fixdt(1, 46, 20)  OutDataTypeStr=fixdt(1, 46, 26)  SaturateOnIntegerOverflow=on  SampleTime=1.62760416666667e-07
  Gain9 : Gain  Gain="fi(0,1,46,78,\"hex\",\"1b7cdfd9d7be\")"  ParamDataTypeStr=fixdt(1, 46, 78)  OutDataTypeStr=fixdt(1, 46, 76)  SaturateOnIntegerOverflow=on  SampleTime=1.62760416666667e-07
  Input_delay{1..5} (5 alike) : Delay  DelayLength=double(1)  InitialCondition=0  SampleTime=1.62760416666667e-07
  Input_delay5_Initial_Val : Constant  OutDataTypeStr=fixdt(0, 4, 0)  SampleTime=1.62760416666667e-07
  Input_delay5_ctrl_const : Constant  OutDataTypeStr=boolean  SampleTime=1.62760416666667e-07
  Input_delay5_ctrl_delay : Delay  DelayLength=double(1)  InitialCondition=0  SampleTime=1.62760416666667e-07
  Input_delay5_switch : Switch  Criteria=u2 ~= 0  Threshold=double(0)  OutDataTypeStr=fixdt(0, 4, 0)  SampleTime=1.62760416666667e-07
  "LUT_Gvar1 " : Lookup_n-D  NumberOfTableDimensions=1  BreakpointsForDimension1="fi(\"numerictype\",numerictype(0,5,0),\"fimath\",fimath(\"RoundingMethod\", \"Nearest\",\"OverflowAction\", \"Saturate\",\"ProductMode\",\"FullPrecision\",\"SumMode\",\"FullPrecision\"),\"Value\",\"[0 1 2 3 4 5 6 7 8 9 10 11 12 13 14 15 16 17 18 19 20 21 22 23 24 25 26 27 28 29 30 31]\")"  Table="reshape(fi(\"numerictype\",numerictype(1,22,30),\"fimath\",fimath(\"RoundingMethod\", \"Floor\",\"OverflowAction\", \"Wrap\",\"ProductMode\",\"FullPrecision\",\"SumMode\",\"FullPrecision\"),\"Value\",\"[0.0013199998065829277039;0.00066000036895275115967;0.00043999962508678436279;0.00033000018447637557983;0.00026400014758110046387;0.0002199998125433921814;0.00018857140094041824341;0.00016499962657690048218;0.0001466665416955947876;0.00013200007379055023193;0.00011999998241662979126;0.00011000037193298339844;0.00010153837502002716064;9.4286166131496429443e-05;8.7999738752841949463e-05;8.2500278949737548828e-05;7.7647157013416290283e-05;7.3333270847797393799e-05;6.947387009859085083e-05;6.6000036895275115967e-05;6.2856823205947875977e-05;6.0000456869602203369e-05;5.7390891015529632568e-05;5.5000185966491699219e-05;5.2800402045249938965e-05;5.0769187510013580322e-05;4.8888847231864929199e-05;4.7142617404460906982e-05;4.5517459511756896973e-05;4.4000335037708282471e-05;4.2580999433994293213e-05;4.1250139474868774414e-05]\"), [1  32])"  InterpMethod=Flat  ExtrapMethod=Clip  DiagnosticForOutOfRangeInput=Error  SampleTime=1.62760416666667e-07  OutDataTypeStr=fixdt(1, 22, 30)  RndMeth=Simplest  InputSameDT=on
  LUT_Gvar2_rev : Lookup_n-D  NumberOfTableDimensions=1  BreakpointsForDimension1="fi(\"numerictype\",numerictype(0,5,0),\"fimath\",fimath(\"RoundingMethod\", \"Nearest\",\"OverflowAction\", \"Saturate\",\"ProductMode\",\"FullPrecision\",\"SumMode\",\"FullPrecision\"),\"Value\",\"[0 1 2 3 4 5 6 7 8 9 10 11 12 13 14 15 16 17 18 19 20 21 22 23 24 25 26 27 28 29 30 31]\")"  Table="reshape(fi(\"numerictype\",numerictype(1,22,29),\"fimath\",fimath(\"RoundingMethod\", \"Floor\",\"OverflowAction\", \"Wrap\",\"ProductMode\",\"FullPrecision\",\"SumMode\",\"FullPrecision\"),\"Value\",\"[0.00010312534868717193604;0.00010645203292369842529;0.00011000037193298339844;0.00011379271745681762695;0.0001178570091724395752;0.00012222304940223693848;0.00012692250311374664307;0.00013200007379055023193;0.00013750046491622924805;0.00014347769320011138916;0.00015000067651271820068;0.00015714205801486968994;0.00016500055789947509766;0.00017368420958518981934;0.00018333271145820617676;0.00019411742687225341797;0.00020625069737434387207;0.00022000074386596679688;0.00023571401834487915039;0.00025384686887264251709;0.00027500092983245849609;0.00029999949038028717041;0.00032999925315380096436;0.00036666728556156158447;0.00041249953210353851318;0.00047142803668975830078;0.00054999999701976776123;0.00066000036895275115967;0.00082500092685222625732;0.0010999999940395355225;0.0016499999910593032837;0.0032999999821186065674]\"), [1  32])"  InterpMethod=Flat  ExtrapMethod=Clip  DiagnosticForOutOfRangeInput=Error  SampleTime=1.62760416666667e-07  OutDataTypeStr=fixdt(1, 22, 29)  RndMeth=Simplest  InputSameDT=on
  "LUT_Gvar3 " : Lookup_n-D  NumberOfTableDimensions=1  BreakpointsForDimension1="fi(\"numerictype\",numerictype(0,5,0),\"fimath\",fimath(\"RoundingMethod\", \"Nearest\",\"OverflowAction\", \"Saturate\",\"ProductMode\",\"FullPrecision\",\"SumMode\",\"FullPrecision\"),\"Value\",\"[0 1 2 3 4 5 6 7 8 9 10 11 12 13 14 15 16 17 18 19 20 21 22 23 24 25 26 27 28 29 30 31]\")"  Table="reshape(fi(\"numerictype\",numerictype(1,22,31),\"fimath\",fimath(\"RoundingMethod\", \"Floor\",\"OverflowAction\", \"Wrap\",\"ProductMode\",\"FullPrecision\",\"SumMode\",\"FullPrecision\"),\"Value\",\"[0.00065999990329146385193;0.00033000018447637557983;0.0002199998125433921814;0.00016500009223818778992;0.00013200007379055023193;0.0001099999062716960907;9.4285700470209121704e-05;8.2499813288450241089e-05;7.3333270847797393799e-05;6.6000036895275115967e-05;5.999999120831489563e-05;5.5000185966491699219e-05;5.0769187510013580322e-05;4.7143083065748214722e-05;4.3999869376420974731e-05;4.1250139474868774414e-05;3.8823578506708145142e-05;3.6666635423898696899e-05;3.4736935049295425415e-05;3.3000018447637557983e-05;3.1428411602973937988e-05;3.0000228434801101685e-05;2.8695445507764816284e-05;2.7500092983245849609e-05;2.6400201022624969482e-05;2.5384593755006790161e-05;2.44444236159324646e-05;2.3571308702230453491e-05;2.2758729755878448486e-05;2.2000167518854141235e-05;2.1290499716997146606e-05;2.0625069737434387207e-05]\"), [1  32])"  InterpMethod=Flat  ExtrapMethod=Clip  DiagnosticForOutOfRangeInput=Error  SampleTime=1.62760416666667e-07  OutDataTypeStr=fixdt(1, 22, 31)  RndMeth=Simplest  InputSameDT=on
  Mult_delay1 : Delay  DelayLength=double(1)  InitialCondition=0  SampleTime=1.62760416666667e-07
  Mult_delay2 : Delay  DelayLength=double(1)  InitialCondition=0  SampleTime=1.62760416666667e-07
  Mult_delay3 : Delay  DelayLength=double(1)  InitialCondition=0  SampleTime=1.62760416666667e-07
  Path Delay {0..5} (6 alike) : Delay  DelayLength=double(1)  InitialCondition=0  SampleTime=1.62760416666667e-07
  Product : Product  Inputs=**  OutDataTypeStr=fixdt(1, 46, 52)  SaturateOnIntegerOverflow=on  SampleTime=1.62760416666667e-07
  Product1 : Product  Inputs=**  OutDataTypeStr=fixdt(1, 46, 52)  SaturateOnIntegerOverflow=on  SampleTime=1.62760416666667e-07
  Product2 : Product  Inputs=**  OutDataTypeStr=fixdt(1, 46, 53)  SaturateOnIntegerOverflow=on  SampleTime=1.62760416666667e-07
  Product3 : Product  Inputs=**  OutDataTypeStr=fixdt(1, 46, 53)  SaturateOnIntegerOverflow=on  SampleTime=1.62760416666667e-07
  Product4 : Product  Inputs=**  OutDataTypeStr=fixdt(1, 46, 51)  SaturateOnIntegerOverflow=on  SampleTime=1.62760416666667e-07
  Product5 : Product  Inputs=**  OutDataTypeStr=fixdt(1, 46, 51)  SaturateOnIntegerOverflow=on  SampleTime=1.62760416666667e-07
  Rate Transition : RateTransition  InitialCondition=double(0)  OutPortSampleTimeOpt=Multiple of input port sample time  OutPortSampleTimeMultiple=1/128
  Rate Transition1 : RateTransition  InitialCondition=double(0)  OutPortSampleTimeOpt=Multiple of input port sample time  OutPortSampleTimeMultiple=128
  Relational Operator4 : RelationalOperator  Operator=>  OutDataTypeStr=boolean  SampleTime=1.62760416666667e-07  RndMeth=Nearest
  Relational Operator7 : RelationalOperator  Operator=<=  OutDataTypeStr=boolean  SampleTime=1.62760416666667e-07  RndMeth=Nearest
  Sum1 : Sum  AccumDataTypeStr=fixdt(0, 5, 0)  OutDataTypeStr=fixdt(0, 4, 0)  SampleTime=1.62760416666667e-07
  Sum10 : Sum  AccumDataTypeStr=fixdt(1, 53, 57)  OutDataTypeStr=fixdt(1, 46, 51)  SaturateOnIntegerOverflow=on  SampleTime=1.62760416666667e-07
  Sum11 : Sum  AccumDataTypeStr=fixdt(1, 49, 54)  OutDataTypeStr=fixdt(1, 46, 52)  SaturateOnIntegerOverflow=on  SampleTime=1.62760416666667e-07
  Sum12 : Sum  AccumDataTypeStr=fixdt(1, 50, 57)  OutDataTypeStr=fixdt(1, 46, 54)  SaturateOnIntegerOverflow=on  SampleTime=1.62760416666667e-07
  Sum13 : Sum  Inputs=+++  AccumDataTypeStr=fixdt(1, 49, 52)  OutDataTypeStr=fixdt(1, 46, 50)  SaturateOnIntegerOverflow=on  SampleTime=1.62760416666667e-07
  Sum14 : Sum  AccumDataTypeStr=fixdt(1, 51, 54)  OutDataTypeStr=fixdt(1, 46, 50)  SaturateOnIntegerOverflow=on  SampleTime=1.62760416666667e-07
  Sum15 : Sum  AccumDataTypeStr=fixdt(1, 49, 53)  OutDataTypeStr=fixdt(1, 46, 51)  SaturateOnIntegerOverflow=on  SampleTime=1.62760416666667e-07
  Sum18 : Sum  AccumDataTypeStr=fixdt(1, 49, 53)  OutDataTypeStr=fixdt(1, 46, 51)  SaturateOnIntegerOverflow=on  SampleTime=1.62760416666667e-07
  Sum2 : Sum  AccumDataTypeStr=fixdt(1, 49, 59)  OutDataTypeStr=fixdt(1, 46, 56)  SaturateOnIntegerOverflow=on  SampleTime=1.62760416666667e-07
  Sum20 : Sum  Inputs=+++  AccumDataTypeStr=fixdt(1, 55, 64)  OutDataTypeStr=fixdt(1, 46, 58)  SaturateOnIntegerOverflow=on  SampleTime=1.62760416666667e-07
  Sum21 : Sum  AccumDataTypeStr=fixdt(1, 51, 60)  OutDataTypeStr=fixdt(1, 46, 56)  SaturateOnIntegerOverflow=on  SampleTime=1.62760416666667e-07
  Sum22 : Sum  AccumDataTypeStr=fixdt(1, 47, 54)  OutDataTypeStr=fixdt(1, 46, 53)  SaturateOnIntegerOverflow=on  SampleTime=1.62760416666667e-07
  Sum23 : Sum  AccumDataTypeStr=fixdt(1, 49, 55)  OutDataTypeStr=fixdt(1, 46, 54)  SaturateOnIntegerOverflow=on  SampleTime=1.62760416666667e-07
  Sum24 : Sum  AccumDataTypeStr=fixdt(1, 49, 55)  OutDataTypeStr=fixdt(1, 46, 54)  SaturateOnIntegerOverflow=on  SampleTime=1.62760416666667e-07
  Sum25 : Sum  AccumDataTypeStr=fixdt(1, 47, 54)  OutDataTypeStr=fixdt(1, 46, 53)  SaturateOnIntegerOverflow=on  SampleTime=1.62760416666667e-07
  Sum28 : Sum  AccumDataTypeStr=fixdt(1, 47, 60)  OutDataTypeStr=fixdt(1, 46, 64)  SaturateOnIntegerOverflow=on  SampleTime=1.62760416666667e-07
  Sum3 : Sum  AccumDataTypeStr=fixdt(1, 54, 63)  OutDataTypeStr=fixdt(1, 46, 56)  SaturateOnIntegerOverflow=on  SampleTime=1.62760416666667e-07
  Sum5 : Sum  AccumDataTypeStr=fixdt(1, 58, 56)  OutDataTypeStr=fixdt(1, 46, 45)  SaturateOnIntegerOverflow=on  SampleTime=1.62760416666667e-07
  Sum6 : Sum  Inputs=+++  AccumDataTypeStr=fixdt(1, 48, 57)  OutDataTypeStr=fixdt(1, 46, 55)  SaturateOnIntegerOverflow=on  SampleTime=1.62760416666667e-07
  Sum7 : Sum  Inputs=+++  AccumDataTypeStr=fixdt(1, 49, 58)  OutDataTypeStr=fixdt(1, 46, 56)  SaturateOnIntegerOverflow=on  SampleTime=1.62760416666667e-07
  Sum8 : Sum  AccumDataTypeStr=fixdt(1, 49, 59)  OutDataTypeStr=fixdt(1, 46, 57)  SaturateOnIntegerOverflow=on  SampleTime=1.62760416666667e-07
  Sum9 : Sum  Inputs=+++  AccumDataTypeStr=fixdt(1, 48, 57)  OutDataTypeStr=fixdt(1, 46, 60)  SaturateOnIntegerOverflow=on  SampleTime=1.62760416666667e-07
  Switch4 : Switch  Criteria=u2 > Threshold  Threshold=double(0)  OutDataTypeStr=fixdt(0, 4, 0)  SampleTime=1.62760416666667e-07
  Switch7 : Switch  Criteria=u2 > Threshold  Threshold=double(0)  OutDataTypeStr=fixdt(0, 4, 0)  SampleTime=1.62760416666667e-07
  To Workspace1 : ToWorkspace  VariableName=input_signal  SaveFormat=Timeseries  SampleTime=1/fs
  To Workspace10 : ToWorkspace  VariableName=opamp_out7  SaveFormat=Timeseries  SampleTime=-1
  To Workspace11 : ToWorkspace  VariableName=opamp_out8  SaveFormat=Timeseries  SampleTime=-1
  To Workspace12 : ToWorkspace  VariableName=opamp_out5  SaveFormat=Timeseries  SampleTime=-1
  To Workspace13 : ToWorkspace  VariableName=Gvar3_N_sim  SaveFormat=Timeseries  SampleTime=1/fs_sim
  To Workspace14 : ToWorkspace  VariableName=Gvar2_N_sim  SaveFormat=Timeseries  SampleTime=1/fs_sim
  To Workspace15 : ToWorkspace  VariableName=Gvar1_N_sim  SaveFormat=Timeseries  SampleTime=1/fs_sim
  To Workspace16 : ToWorkspace  VariableName=Gvar4_N_sim  SaveFormat=Timeseries  SampleTime=1/(fs_sim)
  To Workspace2 : ToWorkspace  VariableName=decicion_comparator  SaveFormat=Timeseries  SampleTime=-1
  To Workspace3 : ToWorkspace  VariableName=output_dem  SaveFormat=Timeseries  SampleTime=-1
  To Workspace4 : ToWorkspace  VariableName=comparator_input_n  SaveFormat=Timeseries  SampleTime=-1
  To Workspace5 : ToWorkspace  VariableName=comparator_input_p  SaveFormat=Timeseries  SampleTime=-1
  To Workspace6 : ToWorkspace  VariableName=delay_line_output  SaveFormat=Timeseries  SampleTime=-1
  To Workspace7 : ToWorkspace  VariableName=opamp_out3  SaveFormat=Timeseries  SampleTime=-1
  To Workspace8 : ToWorkspace  VariableName=opamp_out4  SaveFormat=Timeseries  SampleTime=-1
  To Workspace9 : ToWorkspace  VariableName=opamp_out1  SaveFormat=Timeseries  SampleTime=-1
  Z22_circuit : Subsystem
  Z23_circuit : Subsystem
  Z24_circuit : Subsystem
  Z25_circuit : Subsystem
  adder{,2..4} (4 alike) : Sum  AccumDataTypeStr=fixdt(1, 46, 42)  OutDataTypeStr=fixdt(1, 46, 42)  SaturateOnIntegerOverflow=on  SampleTime=1.62760416666667e-07
  adder1 : Sum  AccumDataTypeStr=fixdt(1, 46, 43)  OutDataTypeStr=fixdt(1, 46, 43)  SaturateOnIntegerOverflow=on  SampleTime=1.62760416666667e-07
  denom_acc1 : Sum  Inputs=+-  AccumDataTypeStr=fixdt(1, 46, 17)  OutDataTypeStr=fixdt(1, 46, 17)  SaturateOnIntegerOverflow=on  SampleTime=1.62760416666667e-07
  denom_acc11 : Sum  Inputs=+-  AccumDataTypeStr=fixdt(1, 46, 40)  OutDataTypeStr=fixdt(1, 46, 40)  SaturateOnIntegerOverflow=on  SampleTime=1.62760416666667e-07
  denom_acc110 : Sum  Inputs=+-  AccumDataTypeStr=fixdt(1, 46, 43)  OutDataTypeStr=fixdt(1, 46, 43)  SaturateOnIntegerOverflow=on  SampleTime=1.62760416666667e-07
  denom_acc111 : Sum  Inputs=+-  AccumDataTypeStr=fixdt(1, 46, 39)  OutDataTypeStr=fixdt(1, 46, 39)  SaturateOnIntegerOverflow=on  SampleTime=1.62760416666667e-07
  denom_acc112 : Sum  Inputs=+-  AccumDataTypeStr=fixdt(1, 46, 47)  OutDataTypeStr=fixdt(1, 46, 47)  SaturateOnIntegerOverflow=on  SampleTime=1.62760416666667e-07
  denom_acc113 : Sum  Inputs=+-  AccumDataTypeStr=fixdt(1, 46, 48)  OutDataTypeStr=fixdt(1, 46, 48)  SaturateOnIntegerOverflow=on  SampleTime=1.62760416666667e-07
  denom_acc114 : Sum  Inputs=+-  AccumDataTypeStr=fixdt(1, 46, 52)  OutDataTypeStr=fixdt(1, 46, 52)  SaturateOnIntegerOverflow=on  SampleTime=1.62760416666667e-07
  denom_acc115 : Sum  Inputs=+-  AccumDataTypeStr=fixdt(1, 46, 26)  OutDataTypeStr=fixdt(1, 46, 26)  SaturateOnIntegerOverflow=on  SampleTime=1.62760416666667e-07
  denom_acc12 : Sum  Inputs=+-  AccumDataTypeStr=fixdt(1, 46, 54)  OutDataTypeStr=fixdt(1, 46, 54)  SaturateOnIntegerOverflow=on  SampleTime=1.62760416666667e-07
  denom_acc13 : Sum  Inputs=+-  AccumDataTypeStr=fixdt(1, 46, 57)  OutDataTypeStr=fixdt(1, 46, 57)  SaturateOnIntegerOverflow=on  SampleTime=1.62760416666667e-07
  denom_acc14 : Sum  Inputs=+-  AccumDataTypeStr=fixdt(1, 46, 40)  OutDataTypeStr=fixdt(1, 46, 40)  SaturateOnIntegerOverflow=on  SampleTime=1.62760416666667e-07
  denom_acc15 : Sum  Inputs=+-  AccumDataTypeStr=fixdt(1, 46, 48)  OutDataTypeStr=fixdt(1, 46, 48)  SaturateOnIntegerOverflow=on  SampleTime=1.62760416666667e-07
  denom_acc16 : Sum  Inputs=+-  AccumDataTypeStr=fixdt(1, 46, 50)  OutDataTypeStr=fixdt(1, 46, 50)  SaturateOnIntegerOverflow=on  SampleTime=1.62760416666667e-07
  denom_acc17 : Sum  Inputs=+-  AccumDataTypeStr=fixdt(1, 46, 57)  OutDataTypeStr=fixdt(1, 46, 57)  SaturateOnIntegerOverflow=on  SampleTime=1.62760416666667e-07
  denom_acc18 : Sum  Inputs=+-  AccumDataTypeStr=fixdt(1, 46, 44)  OutDataTypeStr=fixdt(1, 46, 44)  SaturateOnIntegerOverflow=on  SampleTime=1.62760416666667e-07
  denom_acc19 : Sum  Inputs=+-  AccumDataTypeStr=fixdt(1, 46, 43)  OutDataTypeStr=fixdt(1, 46, 43)  SaturateOnIntegerOverflow=on  SampleTime=1.62760416666667e-07
  denom_acc2 : Sum  Inputs=+-  AccumDataTypeStr=fixdt(1, 46, 17)  OutDataTypeStr=fixdt(1, 46, 17)  SaturateOnIntegerOverflow=on  SampleTime=1.62760416666667e-07
  denom_acc3 : Sum  Inputs=+-  AccumDataTypeStr=fixdt(1, 46, 17)  OutDataTypeStr=fixdt(1, 46, 17)  SaturateOnIntegerOverflow=on  SampleTime=1.62760416666667e-07
  denom_acc_cast1 : DataTypeConversion  OutDataTypeStr=fixdt(1, 46, 17)  SampleTime=1.62760416666667e-07  SaturateOnIntegerOverflow=on
  denom_acc_cast11 : DataTypeConversion  OutDataTypeStr=fixdt(1, 46, 57)  SampleTime=1.62760416666667e-07  SaturateOnIntegerOverflow=on
  denom_acc_cast110 : DataTypeConversion  OutDataTypeStr=fixdt(1, 46, 52)  SampleTime=1.62760416666667e-07  SaturateOnIntegerOverflow=on
  denom_acc_cast111 : DataTypeConversion  OutDataTypeStr=fixdt(1, 46, 48)  SampleTime=1.62760416666667e-07  SaturateOnIntegerOverflow=on
  denom_acc_cast112 : DataTypeConversion  OutDataTypeStr=fixdt(1, 46, 47)  SampleTime=1.62760416666667e-07  SaturateOnIntegerOverflow=on
  denom_acc_cast113 : DataTypeConversion  OutDataTypeStr=fixdt(1, 46, 43)  SampleTime=1.62760416666667e-07  SaturateOnIntegerOverflow=on
  denom_acc_cast114 : DataTypeConversion  OutDataTypeStr=fixdt(1, 46, 39)  SampleTime=1.62760416666667e-07  SaturateOnIntegerOverflow=on
  denom_acc_cast115 : DataTypeConversion  OutDataTypeStr=fixdt(1, 46, 26)  SampleTime=1.62760416666667e-07  SaturateOnIntegerOverflow=on
  denom_acc_cast12 : DataTypeConversion  OutDataTypeStr=fixdt(1, 46, 54)  SampleTime=1.62760416666667e-07  SaturateOnIntegerOverflow=on
  denom_acc_cast13 : DataTypeConversion  OutDataTypeStr=fixdt(1, 46, 40)  SampleTime=1.62760416666667e-07  SaturateOnIntegerOverflow=on
  denom_acc_cast14 : DataTypeConversion  OutDataTypeStr=fixdt(1, 46, 40)  SampleTime=1.62760416666667e-07  SaturateOnIntegerOverflow=on
  denom_acc_cast15 : DataTypeConversion  OutDataTypeStr=fixdt(1, 46, 57)  SampleTime=1.62760416666667e-07  SaturateOnIntegerOverflow=on
  denom_acc_cast16 : DataTypeConversion  OutDataTypeStr=fixdt(1, 46, 50)  SampleTime=1.62760416666667e-07  SaturateOnIntegerOverflow=on
  denom_acc_cast17 : DataTypeConversion  OutDataTypeStr=fixdt(1, 46, 48)  SampleTime=1.62760416666667e-07  SaturateOnIntegerOverflow=on
  denom_acc_cast18 : DataTypeConversion  OutDataTypeStr=fixdt(1, 46, 44)  SampleTime=1.62760416666667e-07  SaturateOnIntegerOverflow=on
  denom_acc_cast19 : DataTypeConversion  OutDataTypeStr=fixdt(1, 46, 43)  SampleTime=1.62760416666667e-07  SaturateOnIntegerOverflow=on
  denom_acc_cast2 : DataTypeConversion  OutDataTypeStr=fixdt(1, 46, 17)  SampleTime=1.62760416666667e-07  SaturateOnIntegerOverflow=on
  denom_acc_cast3 : DataTypeConversion  OutDataTypeStr=fixdt(1, 46, 17)  SampleTime=1.62760416666667e-07  SaturateOnIntegerOverflow=on
  denom_gain1 : Gain  Gain="fi(0,1,19,16,\"hex\",\"54598\")"  ParamDataTypeStr=fixdt(1, 19, 16)  OutDataTypeStr=fixdt(1, 46, 17)  SaturateOnIntegerOverflow=on  SampleTime=1.62760416666667e-07
  denom_gain11 : Gain  Gain="fi(0,1,17,15,\"hex\",\"18443\")"  ParamDataTypeStr=fixdt(1, 17, 15)  OutDataTypeStr=fixdt(1, 46, 57)  SaturateOnIntegerOverflow=on  SampleTime=1.62760416666667e-07
  denom_gain110 : Gain  Gain="fi(0,1,17,15,\"hex\",\"18287\")"  ParamDataTypeStr=fixdt(1, 17, 15)  OutDataTypeStr=fixdt(1, 46, 52)  SaturateOnIntegerOverflow=on  SampleTime=1.62760416666667e-07
  denom_gain111 : Gain  Gain="fi(0,1,15,13,\"hex\",\"6019\")"  ParamDataTypeStr=fixdt(1, 15, 13)  OutDataTypeStr=fixdt(1, 46, 48)  SaturateOnIntegerOverflow=on  SampleTime=1.62760416666667e-07
  denom_gain112 : Gain  Gain="fi(0,1,18,16,\"hex\",\"300e7\")"  ParamDataTypeStr=fixdt(1, 18, 16)  OutDataTypeStr=fixdt(1, 46, 47)  SaturateOnIntegerOverflow=on  SampleTime=1.62760416666667e-07
  denom_gain113 : Gain  Gain="fi(0,1,18,16,\"hex\",\"30005\")"  ParamDataTypeStr=fixdt(1, 18, 16)  OutDataTypeStr=fixdt(1, 46, 43)  SaturateOnIntegerOverflow=on  SampleTime=1.62760416666667e-07
  denom_gain114 : Gain  Gain="fi(0,1,18,16,\"hex\",\"30001\")"  ParamDataTypeStr=fixdt(1, 18, 16)  OutDataTypeStr=fixdt(1, 46, 39)  SaturateOnIntegerOverflow=on  SampleTime=1.62760416666667e-07
  denom_gain115 : Gain  Gain="fi(0,1,24,22,\"hex\",\"c00007\")"  ParamDataTypeStr=fixdt(1, 24, 22)  OutDataTypeStr=fixdt(1, 46, 26)  SaturateOnIntegerOverflow=on  SampleTime=1.62760416666667e-07
  denom_gain12 : Gain  Gain="fi(0,1,18,16,\"hex\",\"347ab\")"  ParamDataTypeStr=fixdt(1, 18, 16)  OutDataTypeStr=fixdt(1, 46, 54)  SaturateOnIntegerOverflow=on  SampleTime=1.62760416666667e-07
  denom_gain13 : Gain  Gain="fi(0,1,18,16,\"hex\",\"30001\")"  ParamDataTypeStr=fixdt(1, 18, 16)  OutDataTypeStr=fixdt(1, 46, 40)  SaturateOnIntegerOverflow=on  SampleTime=1.62760416666667e-07
  denom_gain14 : Gain  Gain="fi(0,1,16,14,\"hex\",\"c001\")"  ParamDataTypeStr=fixdt(1, 16, 14)  OutDataTypeStr=fixdt(1, 46, 40)  SaturateOnIntegerOverflow=on  SampleTime=1.62760416666667e-07
  denom_gain15 : Gain  Gain="fi(0,1,18,16,\"hex\",\"30373\")"  ParamDataTypeStr=fixdt(1, 18, 16)  OutDataTypeStr=fixdt(1, 46, 57)  SaturateOnIntegerOverflow=on  SampleTime=1.62760416666667e-07
  denom_gain16 : Gain  Gain="fi(0,1,17,15,\"hex\",\"18071\")"  ParamDataTypeStr=fixdt(1, 17, 15)  OutDataTypeStr=fixdt(1, 46, 50)  SaturateOnIntegerOverflow=on  SampleTime=1.62760416666667e-07
  denom_gain17 : Gain  Gain="fi(0,1,17,15,\"hex\",\"18059\")"  ParamDataTypeStr=fixdt(1, 17, 15)  OutDataTypeStr=fixdt(1, 46, 48)  SaturateOnIntegerOverflow=on  SampleTime=1.62760416666667e-07
  denom_gain18 : Gain  Gain="fi(0,1,17,15,\"hex\",\"18011\")"  ParamDataTypeStr=fixdt(1, 17, 15)  OutDataTypeStr=fixdt(1, 46, 44)  SaturateOnIntegerOverflow=on  SampleTime=1.62760416666667e-07
  denom_gain19 : Gain  Gain="fi(0,1,18,16,\"hex\",\"3000f\")"  ParamDataTypeStr=fixdt(1, 18, 16)  OutDataTypeStr=fixdt(1, 46, 43)  SaturateOnIntegerOverflow=on  SampleTime=1.62760416666667e-07
  denom_gain2 : Gain  Gain="fi(0,1,19,16,\"hex\",\"276f1\")"  ParamDataTypeStr=fixdt(1, 19, 16)  OutDataTypeStr=fixdt(1, 46, 17)  SaturateOnIntegerOverflow=on  SampleTime=1.62760416666667e-07
  denom_gain3 : Gain  Gain="fi(0,1,19,16,\"hex\",\"74377\")"  ParamDataTypeStr=fixdt(1, 19, 16)  OutDataTypeStr=fixdt(1, 46, 17)  SaturateOnIntegerOverflow=on  SampleTime=1.62760416666667e-07
  denom_scale_by_a0 : hdlmdlgenlib/Buffer
      settings: SourceProductBaseCode=SL
  denom_scale_by_a01 : hdlmdlgenlib/Buffer
      settings: SourceProductBaseCode=SL
  denom_scale_by_a010 : hdlmdlgenlib/Buffer
      settings: SourceProductBaseCode=SL
  denom_scale_by_a011 : hdlmdlgenlib/Buffer
      settings: SourceProductBaseCode=SL
  denom_scale_by_a012 : hdlmdlgenlib/Buffer
      settings: SourceProductBaseCode=SL
  denom_scale_by_a013 : hdlmdlgenlib/Buffer
      settings: SourceProductBaseCode=SL
  denom_scale_by_a014 : hdlmdlgenlib/Buffer
      settings: SourceProductBaseCode=SL
  denom_scale_by_a015 : hdlmdlgenlib/Buffer
      settings: SourceProductBaseCode=SL
  denom_scale_by_a02 : hdlmdlgenlib/Buffer
      settings: SourceProductBaseCode=SL
  denom_scale_by_a03 : hdlmdlgenlib/Buffer
      settings: SourceProductBaseCode=SL
  denom_scale_by_a04 : hdlmdlgenlib/Buffer
      settings: SourceProductBaseCode=SL
  denom_scale_by_a05 : hdlmdlgenlib/Buffer
      settings: SourceProductBaseCode=SL
  denom_scale_by_a06 : hdlmdlgenlib/Buffer
      settings: SourceProductBaseCode=SL
  denom_scale_by_a07 : hdlmdlgenlib/Buffer
      settings: SourceProductBaseCode=SL
  denom_scale_by_a08 : hdlmdlgenlib/Buffer
      settings: SourceProductBaseCode=SL
  denom_scale_by_a09 : hdlmdlgenlib/Buffer
      settings: SourceProductBaseCode=SL
  dtc{,2,4,6,8} (5 alike) : DataTypeConversion  OutDataTypeStr=fixdt(1, 46, 0)  ConvertRealWorld=Stored Integer (SI)  SampleTime=1.62760416666667e-07  SaturateOnIntegerOverflow=on
  dtc{1,5,7,9} (4 alike) : DataTypeConversion  OutDataTypeStr=fixdt(1, 46, 42)  ConvertRealWorld=Stored Integer (SI)  SampleTime=1.62760416666667e-07  SaturateOnIntegerOverflow=on
  dtc3 : DataTypeConversion  OutDataTypeStr=fixdt(1, 46, 43)  ConvertRealWorld=Stored Integer (SI)  SampleTime=1.62760416666667e-07  SaturateOnIntegerOverflow=on
  gain : Gain  Gain="fi(0,1,46,51,\"hex\",\"15d867c3ece3\")"  ParamDataTypeStr=fixdt(1, 46, 51)  OutDataTypeStr=fixdt(1, 46, 0)  SaturateOnIntegerOverflow=on  SampleTime=1.62760416666667e-07
  gain1 : Gain  Gain="fi(0,1,46,54,\"hex\",\"15d867c3ece3\")"  ParamDataTypeStr=fixdt(1, 46, 54)  OutDataTypeStr=fixdt(1, 46, 0)  SaturateOnIntegerOverflow=on  SampleTime=1.62760416666667e-07
  gain2 : Gain  Gain="fi(0,1,46,48,\"hex\",\"15d867c3ece3\")"  ParamDataTypeStr=fixdt(1, 46, 48)  OutDataTypeStr=fixdt(1, 46, 0)  SaturateOnIntegerOverflow=on  SampleTime=1.62760416666667e-07
  gain3 : Gain  Gain="fi(0,1,46,48,\"hex\",\"15d867c3ece3\")"  ParamDataTypeStr=fixdt(1, 46, 48)  OutDataTypeStr=fixdt(1, 46, 0)  SaturateOnIntegerOverflow=on  SampleTime=1.62760416666667e-07
  gain4 : Gain  Gain="fi(0,1,46,49,\"hex\",\"15d867c3ece3\")"  ParamDataTypeStr=fixdt(1, 46, 49)  OutDataTypeStr=fixdt(1, 46, 0)  SaturateOnIntegerOverflow=on  SampleTime=1.62760416666667e-07
  input_acc_cast : DataTypeConversion  OutDataTypeStr=fixdt(1, 46, 17)  SampleTime=1.62760416666667e-07  SaturateOnIntegerOverflow=on
  input_acc_cast1 : DataTypeConversion  OutDataTypeStr=fixdt(1, 46, 40)  SampleTime=1.62760416666667e-07  SaturateOnIntegerOverflow=on
  input_acc_cast10 : DataTypeConversion  OutDataTypeStr=fixdt(1, 46, 43)  SampleTime=1.62760416666667e-07  SaturateOnIntegerOverflow=on
  input_acc_cast11 : DataTypeConversion  OutDataTypeStr=fixdt(1, 46, 39)  SampleTime=1.62760416666667e-07  SaturateOnIntegerOverflow=on
  input_acc_cast12 : DataTypeConversion  OutDataTypeStr=fixdt(1, 46, 47)  SampleTime=1.62760416666667e-07  SaturateOnIntegerOverflow=on
  input_acc_cast13 : DataTypeConversion  OutDataTypeStr=fixdt(1, 46, 48)  SampleTime=1.62760416666667e-07  SaturateOnIntegerOverflow=on
  input_acc_cast14 : DataTypeConversion  OutDataTypeStr=fixdt(1, 46, 52)  SampleTime=1.62760416666667e-07  SaturateOnIntegerOverflow=on
  input_acc_cast15 : DataTypeConversion  OutDataTypeStr=fixdt(1, 46, 26)  SampleTime=1.62760416666667e-07  SaturateOnIntegerOverflow=on
  input_acc_cast2 : DataTypeConversion  OutDataTypeStr=fixdt(1, 46, 54)  SampleTime=1.62760416666667e-07  SaturateOnIntegerOverflow=on
  input_acc_cast3 : DataTypeConversion  OutDataTypeStr=fixdt(1, 46, 57)  SampleTime=1.62760416666667e-07  SaturateOnIntegerOverflow=on
  input_acc_cast4 : DataTypeConversion  OutDataTypeStr=fixdt(1, 46, 40)  SampleTime=1.62760416666667e-07  SaturateOnIntegerOverflow=on
  input_acc_cast5 : DataTypeConversion  OutDataTypeStr=fixdt(1, 46, 48)  SampleTime=1.62760416666667e-07  SaturateOnIntegerOverflow=on
  input_acc_cast6 : DataTypeConversion  OutDataTypeStr=fixdt(1, 46, 50)  SampleTime=1.62760416666667e-07  SaturateOnIntegerOverflow=on
  input_acc_cast7 : DataTypeConversion  OutDataTypeStr=fixdt(1, 46, 57)  SampleTime=1.62760416666667e-07  SaturateOnIntegerOverflow=on
  input_acc_cast8 : DataTypeConversion  OutDataTypeStr=fixdt(1, 46, 44)  SampleTime=1.62760416666667e-07  SaturateOnIntegerOverflow=on
  input_acc_cast9 : DataTypeConversion  OutDataTypeStr=fixdt(1, 46, 43)  SampleTime=1.62760416666667e-07  SaturateOnIntegerOverflow=on
  nume_acc_cast1 : DataTypeConversion  OutDataTypeStr=fixdt(1, 46, 25)  SampleTime=1.62760416666667e-07  SaturateOnIntegerOverflow=on
  nume_acc_cast11 : DataTypeConversion  OutDataTypeStr=fixdt(1, 46, 50)  SampleTime=1.62760416666667e-07  SaturateOnIntegerOverflow=on
  nume_acc_cast{12,17,110..111} (4 alike) : DataTypeConversion  OutDataTypeStr=fixdt(1, 46, 44)  SampleTime=1.62760416666667e-07  SaturateOnIntegerOverflow=on
  nume_acc_cast{13..14,18..19,112..113} (6 alike) : DataTypeConversion  OutDataTypeStr=fixdt(1, 46, 43)  SampleTime=1.62760416666667e-07  SaturateOnIntegerOverflow=on
  nume_acc_cast114 : DataTypeConversion  OutDataTypeStr=fixdt(1, 46, 42)  SampleTime=1.62760416666667e-07  SaturateOnIntegerOverflow=on
  nume_acc_cast15 : DataTypeConversion  OutDataTypeStr=fixdt(1, 46, 50)  SampleTime=1.62760416666667e-07  SaturateOnIntegerOverflow=on
  nume_acc_cast16 : DataTypeConversion  OutDataTypeStr=fixdt(1, 46, 46)  SampleTime=1.62760416666667e-07  SaturateOnIntegerOverflow=on
  nume_acc_cast2 : DataTypeConversion  OutDataTypeStr=fixdt(1, 46, 25)  SampleTime=1.62760416666667e-07  SaturateOnIntegerOverflow=on
  nume_acc_cast3 : DataTypeConversion  OutDataTypeStr=fixdt(1, 46, 25)  SampleTime=1.62760416666667e-07  SaturateOnIntegerOverflow=on
  nume_gain1 : Gain  Gain="fi(0,1,17,23,\"hex\",\"17aa9\")"  ParamDataTypeStr=fixdt(1, 17, 23)  OutDataTypeStr=fixdt(1, 46, 26)  SaturateOnIntegerOverflow=on  SampleTime=1.62760416666667e-07
  nume_gain11 : Gain  Gain="fi(0,1,10,2,\"hex\",\"123\")"  ParamDataTypeStr=fixdt(1, 10, 2)  OutDataTypeStr=fixdt(1, 46, 51)  SaturateOnIntegerOverflow=on  SampleTime=1.62760416666667e-07
  nume_gain110 : Gain  Gain="fi(0,1,16,8,\"hex\",\"767f\")"  ParamDataTypeStr=fixdt(1, 16, 8)  OutDataTypeStr=fixdt(1, 46, 45)  SaturateOnIntegerOverflow=on  SampleTime=1.62760416666667e-07
  nume_gain111 : Gain  Gain="fi(0,1,18,13,\"hex\",\"10405\")"  ParamDataTypeStr=fixdt(1, 18, 13)  OutDataTypeStr=fixdt(1, 46, 45)  SaturateOnIntegerOverflow=on  SampleTime=1.62760416666667e-07
  nume_gain112 : Gain  Gain="fi(0,1,18,13,\"hex\",\"103f5\")"  ParamDataTypeStr=fixdt(1, 18, 13)  OutDataTypeStr=fixdt(1, 46, 44)  SaturateOnIntegerOverflow=on  SampleTime=1.62760416666667e-07
  nume_gain113 : Gain  Gain="fi(0,1,17,16,\"hex\",\"0d053\")"  ParamDataTypeStr=fixdt(1, 17, 16)  OutDataTypeStr=fixdt(1, 46, 44)  SaturateOnIntegerOverflow=on  SampleTime=1.62760416666667e-07
  nume_gain114 : Gain  Gain="fi(0,1,16,18,\"hex\",\"5355\")"  ParamDataTypeStr=fixdt(1, 16, 18)  OutDataTypeStr=fixdt(1, 46, 43)  SaturateOnIntegerOverflow=on  SampleTime=1.62760416666667e-07
  nume_gain115 : Gain  Gain="fi(0,1,20,19,\"hex\",\"80995\")"  ParamDataTypeStr=fixdt(1, 20, 19)  OutDataTypeStr=fixdt(1, 46, 26)  SaturateOnIntegerOverflow=on  SampleTime=1.62760416666667e-07
  nume_gain12 : Gain  Gain="fi(0,1,17,6,\"hex\",\"0aef9\")"  ParamDataTypeStr=fixdt(1, 17, 6)  OutDataTypeStr=fixdt(1, 46, 45)  SaturateOnIntegerOverflow=on  SampleTime=1.62760416666667e-07
  nume_gain13 : Gain  Gain="fi(0,1,16,18,\"hex\",\"5355\")"  ParamDataTypeStr=fixdt(1, 16, 18)  OutDataTypeStr=fixdt(1, 46, 44)  SaturateOnIntegerOverflow=on  SampleTime=1.62760416666667e-07
  nume_gain14 : Gain  Gain="fi(0,1,17,19,\"hex\",\"0a503\")"  ParamDataTypeStr=fixdt(1, 17, 19)  OutDataTypeStr=fixdt(1, 46, 44)  SaturateOnIntegerOverflow=on  SampleTime=1.62760416666667e-07
  nume_gain15 : Gain  Gain="fi(0,1,16,8,\"hex\",\"50d5\")"  ParamDataTypeStr=fixdt(1, 16, 8)  OutDataTypeStr=fixdt(1, 46, 51)  SaturateOnIntegerOverflow=on  SampleTime=1.62760416666667e-07
  nume_gain16 : Gain  Gain="fi(0,1,15,10,\"hex\",\"207f\")"  ParamDataTypeStr=fixdt(1, 15, 10)  OutDataTypeStr=fixdt(1, 46, 47)  SaturateOnIntegerOverflow=on  SampleTime=1.62760416666667e-07
  nume_gain17 : Gain  Gain="fi(0,1,14,9,\"hex\",\"1041\")"  ParamDataTypeStr=fixdt(1, 14, 9)  OutDataTypeStr=fixdt(1, 46, 45)  SaturateOnIntegerOverflow=on  SampleTime=1.62760416666667e-07
  nume_gain18 : Gain  Gain="fi(0,1,16,14,\"hex\",\"4c93\")"  ParamDataTypeStr=fixdt(1, 16, 14)  OutDataTypeStr=fixdt(1, 46, 44)  SaturateOnIntegerOverflow=on  SampleTime=1.62760416666667e-07
  nume_gain19 : Gain  Gain="fi(0,1,18,17,\"hex\",\"115bf\")"  ParamDataTypeStr=fixdt(1, 18, 17)  OutDataTypeStr=fixdt(1, 46, 44)  SaturateOnIntegerOverflow=on  SampleTime=1.62760416666667e-07
  nume_gain2 : Gain  Gain="fi(0,1,17,23,\"hex\",\"08557\")"  ParamDataTypeStr=fixdt(1, 17, 23)  OutDataTypeStr=fixdt(1, 46, 26)  SaturateOnIntegerOverflow=on  SampleTime=1.62760416666667e-07
  nume_gain3 : Gain  Gain="fi(0,1,17,23,\"hex\",\"08557\")"  ParamDataTypeStr=fixdt(1, 17, 23)  OutDataTypeStr=fixdt(1, 46, 26)  SaturateOnIntegerOverflow=on  SampleTime=1.62760416666667e-07
  nume_gain_b0 : Gain  Gain="fi(0,1,17,23,\"hex\",\"17aa9\")"  ParamDataTypeStr=fixdt(1, 17, 23)  OutDataTypeStr=fixdt(1, 46, 26)  SaturateOnIntegerOverflow=on  SampleTime=1.62760416666667e-07
  nume_gain_b01 : Gain  Gain="fi(0,1,16,18,\"hex\",\"5355\")"  ParamDataTypeStr=fixdt(1, 16, 18)  OutDataTypeStr=fixdt(1, 46, 44)  SaturateOnIntegerOverflow=on  SampleTime=1.62760416666667e-07
  nume_gain_b010 : Gain  Gain="fi(0,1,17,16,\"hex\",\"0d053\")"  ParamDataTypeStr=fixdt(1, 17, 16)  OutDataTypeStr=fixdt(1, 46, 44)  SaturateOnIntegerOverflow=on  SampleTime=1.62760416666667e-07
  nume_gain_b011 : Gain  Gain="fi(0,1,16,18,\"hex\",\"5355\")"  ParamDataTypeStr=fixdt(1, 16, 18)  OutDataTypeStr=fixdt(1, 46, 43)  SaturateOnIntegerOverflow=on  SampleTime=1.62760416666667e-07
  nume_gain_b012 : Gain  Gain="fi(0,1,18,13,\"hex\",\"103f5\")"  ParamDataTypeStr=fixdt(1, 18, 13)  OutDataTypeStr=fixdt(1, 46, 44)  SaturateOnIntegerOverflow=on  SampleTime=1.62760416666667e-07
  nume_gain_b013 : Gain  Gain="fi(0,1,18,13,\"hex\",\"10405\")"  ParamDataTypeStr=fixdt(1, 18, 13)  OutDataTypeStr=fixdt(1, 46, 45)  SaturateOnIntegerOverflow=on  SampleTime=1.62760416666667e-07
  nume_gain_b014 : Gain  Gain="fi(0,1,16,8,\"hex\",\"767f\")"  ParamDataTypeStr=fixdt(1, 16, 8)  OutDataTypeStr=fixdt(1, 46, 45)  SaturateOnIntegerOverflow=on  SampleTime=1.62760416666667e-07
  nume_gain_b015 : Gain  Gain="fi(0,1,20,19,\"hex\",\"7f66b\")"  ParamDataTypeStr=fixdt(1, 20, 19)  OutDataTypeStr=fixdt(1, 46, 26)  SaturateOnIntegerOverflow=on  SampleTime=1.62760416666667e-07
  nume_gain_b02 : Gain  Gain="fi(0,1,17,6,\"hex\",\"0aef9\")"  ParamDataTypeStr=fixdt(1, 17, 6)  OutDataTypeStr=fixdt(1, 46, 45)  SaturateOnIntegerOverflow=on  SampleTime=1.62760416666667e-07
  nume_gain_b03 : Gain  Gain="fi(0,1,10,2,\"hex\",\"123\")"  ParamDataTypeStr=fixdt(1, 10, 2)  OutDataTypeStr=fixdt(1, 46, 51)  SaturateOnIntegerOverflow=on  SampleTime=1.62760416666667e-07
  nume_gain_b04 : Gain  Gain="fi(0,1,17,19,\"hex\",\"0a503\")"  ParamDataTypeStr=fixdt(1, 17, 19)  OutDataTypeStr=fixdt(1, 46, 44)  SaturateOnIntegerOverflow=on  SampleTime=1.62760416666667e-07
  nume_gain_b05 : Gain  Gain="fi(0,1,14,9,\"hex\",\"1041\")"  ParamDataTypeStr=fixdt(1, 14, 9)  OutDataTypeStr=fixdt(1, 46, 45)  SaturateOnIntegerOverflow=on  SampleTime=1.62760416666667e-07
  nume_gain_b06 : Gain  Gain="fi(0,1,15,10,\"hex\",\"207f\")"  ParamDataTypeStr=fixdt(1, 15, 10)  OutDataTypeStr=fixdt(1, 46, 47)  SaturateOnIntegerOverflow=on  SampleTime=1.62760416666667e-07
  nume_gain_b07 : Gain  Gain="fi(0,1,16,8,\"hex\",\"50d5\")"  ParamDataTypeStr=fixdt(1, 16, 8)  OutDataTypeStr=fixdt(1, 46, 51)  SaturateOnIntegerOverflow=on  SampleTime=1.62760416666667e-07
  nume_gain_b08 : Gain  Gain="fi(0,1,16,14,\"hex\",\"4c93\")"  ParamDataTypeStr=fixdt(1, 16, 14)  OutDataTypeStr=fixdt(1, 46, 44)  SaturateOnIntegerOverflow=on  SampleTime=1.62760416666667e-07
  nume_gain_b09 : Gain  Gain="fi(0,1,18,17,\"hex\",\"115bf\")"  ParamDataTypeStr=fixdt(1, 18, 17)  OutDataTypeStr=fixdt(1, 46, 44)  SaturateOnIntegerOverflow=on  SampleTime=1.62760416666667e-07
  nume_gain_b0_cast : DataTypeConversion  OutDataTypeStr=fixdt(1, 46, 25)  SampleTime=1.62760416666667e-07  SaturateOnIntegerOverflow=on
  nume_gain_b0_cast{1,4,8..10,12} (6 alike) : DataTypeConversion  OutDataTypeStr=fixdt(1, 46, 43)  SampleTime=1.62760416666667e-07  SaturateOnIntegerOverflow=on
  nume_gain_b0_cast11 : DataTypeConversion  OutDataTypeStr=fixdt(1, 46, 42)  SampleTime=1.62760416666667e-07  SaturateOnIntegerOverflow=on
  nume_gain_b0_cast{2,5,13..14} (4 alike) : DataTypeConversion  OutDataTypeStr=fixdt(1, 46, 44)  SampleTime=1.62760416666667e-07  SaturateOnIntegerOverflow=on
  nume_gain_b0_cast3 : DataTypeConversion  OutDataTypeStr=fixdt(1, 46, 50)  SampleTime=1.62760416666667e-07  SaturateOnIntegerOverflow=on
  nume_gain_b0_cast6 : DataTypeConversion  OutDataTypeStr=fixdt(1, 46, 46)  SampleTime=1.62760416666667e-07  SaturateOnIntegerOverflow=on
  nume_gain_b0_cast7 : DataTypeConversion  OutDataTypeStr=fixdt(1, 46, 50)  SampleTime=1.62760416666667e-07  SaturateOnIntegerOverflow=on
  output_cast{,1,4,8..10,12,15} (8 alike) : DataTypeConversion  OutDataTypeStr=fixdt(1, 46, 43)  SampleTime=1.62760416666667e-07  SaturateOnIntegerOverflow=on
  output_cast11 : DataTypeConversion  OutDataTypeStr=fixdt(1, 46, 42)  SampleTime=1.62760416666667e-07  SaturateOnIntegerOverflow=on
  output_cast{2,5,13..14} (4 alike) : DataTypeConversion  OutDataTypeStr=fixdt(1, 46, 44)  SampleTime=1.62760416666667e-07  SaturateOnIntegerOverflow=on
  output_cast3 : DataTypeConversion  OutDataTypeStr=fixdt(1, 46, 50)  SampleTime=1.62760416666667e-07  SaturateOnIntegerOverflow=on
  output_cast6 : DataTypeConversion  OutDataTypeStr=fixdt(1, 46, 46)  SampleTime=1.62760416666667e-07  SaturateOnIntegerOverflow=on
  output_cast7 : DataTypeConversion  OutDataTypeStr=fixdt(1, 46, 50)  SampleTime=1.62760416666667e-07  SaturateOnIntegerOverflow=on
  s_nume_acc1 : Sum  OutDataTypeStr=fixdt(1, 46, 25)  SaturateOnIntegerOverflow=on  SampleTime=1.62760416666667e-07
  s_nume_acc{11,14,18..19,110,112} (6 alike) : Sum  OutDataTypeStr=fixdt(1, 46, 43)  SaturateOnIntegerOverflow=on  SampleTime=1.62760416666667e-07
  s_nume_acc111 : Sum  OutDataTypeStr=fixdt(1, 46, 42)  SaturateOnIntegerOverflow=on  SampleTime=1.62760416666667e-07
  s_nume_acc{12,15,113..114} (4 alike) : Sum  OutDataTypeStr=fixdt(1, 46, 44)  SaturateOnIntegerOverflow=on  SampleTime=1.62760416666667e-07
  s_nume_acc115 : Sum  OutDataTypeStr=fixdt(1, 46, 26)  SaturateOnIntegerOverflow=on  SampleTime=1.62760416666667e-07
  s_nume_acc13 : Sum  OutDataTypeStr=fixdt(1, 46, 50)  SaturateOnIntegerOverflow=on  SampleTime=1.62760416666667e-07
  s_nume_acc16 : Sum  OutDataTypeStr=fixdt(1, 46, 46)  SaturateOnIntegerOverflow=on  SampleTime=1.62760416666667e-07
  s_nume_acc17 : Sum  OutDataTypeStr=fixdt(1, 46, 50)  SaturateOnIntegerOverflow=on  SampleTime=1.62760416666667e-07
  s_nume_acc2 : Sum  OutDataTypeStr=fixdt(1, 46, 25)  SaturateOnIntegerOverflow=on  SampleTime=1.62760416666667e-07
  s_nume_acc3 : Sum  OutDataTypeStr=fixdt(1, 46, 25)  SaturateOnIntegerOverflow=on  SampleTime=1.62760416666667e-07
  s_output_cast_wire{,1..13} (14 alike) : hdlmdlgenlib/Buffer
      settings: SourceProductBaseCode=SL
  s_state_out1 : UnitDelay  InitialCondition="fi(0,1,46,18,\"hex\",\"000000000000\")"  SampleTime=1.62760416666667e-07
  s_state_out11 : UnitDelay  InitialCondition="fi(0,1,46,26,\"hex\",\"000000000000\")"  SampleTime=1.62760416666667e-07
  s_state_out110 : UnitDelay  InitialCondition="fi(0,1,46,40,\"hex\",\"000000000000\")"  SampleTime=1.62760416666667e-07
  s_state_out111 : UnitDelay  InitialCondition="fi(0,1,46,50,\"hex\",\"000000000000\")"  SampleTime=1.62760416666667e-07
  s_state_out112 : UnitDelay  InitialCondition="fi(0,1,46,48,\"hex\",\"000000000000\")"  SampleTime=1.62760416666667e-07
  s_state_out113 : UnitDelay  InitialCondition="fi(0,1,46,57,\"hex\",\"000000000000\")"  SampleTime=1.62760416666667e-07
  s_state_out114 : UnitDelay  InitialCondition="fi(0,1,46,39,\"hex\",\"000000000000\")"  SampleTime=1.62760416666667e-07
  s_state_out115 : UnitDelay  InitialCondition="fi(0,1,46,47,\"hex\",\"000000000000\")"  SampleTime=1.62760416666667e-07
  s_state_out12 : UnitDelay  InitialCondition="fi(0,1,46,43,\"hex\",\"000000000000\")"  SampleTime=1.62760416666667e-07
  s_state_out13 : UnitDelay  InitialCondition="fi(0,1,46,44,\"hex\",\"000000000000\")"  SampleTime=1.62760416666667e-07
  s_state_out14 : UnitDelay  InitialCondition="fi(0,1,46,57,\"hex\",\"000000000000\")"  SampleTime=1.62760416666667e-07
  s_state_out15 : UnitDelay  InitialCondition="fi(0,1,46,52,\"hex\",\"000000000000\")"  SampleTime=1.62760416666667e-07
  s_state_out16 : UnitDelay  InitialCondition="fi(0,1,46,48,\"hex\",\"000000000000\")"  SampleTime=1.62760416666667e-07
  s_state_out17 : UnitDelay  InitialCondition="fi(0,1,46,43,\"hex\",\"000000000000\")"  SampleTime=1.62760416666667e-07
  s_state_out18 : UnitDelay  InitialCondition="fi(0,1,46,54,\"hex\",\"000000000000\")"  SampleTime=1.62760416666667e-07
  s_state_out19 : UnitDelay  InitialCondition="fi(0,1,46,40,\"hex\",\"000000000000\")"  SampleTime=1.62760416666667e-07
  s_state_out2 : UnitDelay  InitialCondition="fi(0,1,46,18,\"hex\",\"000000000000\")"  SampleTime=1.62760416666667e-07
  s_state_out3 : UnitDelay  InitialCondition="fi(0,1,46,18,\"hex\",\"000000000000\")"  SampleTime=1.62760416666667e-07
  state_cast : DataTypeConversion  OutDataTypeStr=fixdt(1, 46, 18)  SampleTime=1.62760416666667e-07  SaturateOnIntegerOverflow=on
  state_cast1 : DataTypeConversion  OutDataTypeStr=fixdt(1, 46, 40)  SampleTime=1.62760416666667e-07  SaturateOnIntegerOverflow=on
  state_cast10 : DataTypeConversion  OutDataTypeStr=fixdt(1, 46, 43)  SampleTime=1.62760416666667e-07  SaturateOnIntegerOverflow=on
  state_cast11 : DataTypeConversion  OutDataTypeStr=fixdt(1, 46, 39)  SampleTime=1.62760416666667e-07  SaturateOnIntegerOverflow=on
  state_cast12 : DataTypeConversion  OutDataTypeStr=fixdt(1, 46, 47)  SampleTime=1.62760416666667e-07  SaturateOnIntegerOverflow=on
  state_cast13 : DataTypeConversion  OutDataTypeStr=fixdt(1, 46, 48)  SampleTime=1.62760416666667e-07  SaturateOnIntegerOverflow=on
  state_cast14 : DataTypeConversion  OutDataTypeStr=fixdt(1, 46, 52)  SampleTime=1.62760416666667e-07  SaturateOnIntegerOverflow=on
  state_cast15 : DataTypeConversion  OutDataTypeStr=fixdt(1, 46, 26)  SampleTime=1.62760416666667e-07  SaturateOnIntegerOverflow=on
  state_cast2 : DataTypeConversion  OutDataTypeStr=fixdt(1, 46, 54)  SampleTime=1.62760416666667e-07  SaturateOnIntegerOverflow=on
  state_cast3 : DataTypeConversion  OutDataTypeStr=fixdt(1, 46, 57)  SampleTime=1.62760416666667e-07  SaturateOnIntegerOverflow=on
  state_cast4 : DataTypeConversion  OutDataTypeStr=fixdt(1, 46, 40)  SampleTime=1.62760416666667e-07  SaturateOnIntegerOverflow=on
  state_cast5 : DataTypeConversion  OutDataTypeStr=fixdt(1, 46, 48)  SampleTime=1.62760416666667e-07  SaturateOnIntegerOverflow=on
  state_cast6 : DataTypeConversion  OutDataTypeStr=fixdt(1, 46, 50)  SampleTime=1.62760416666667e-07  SaturateOnIntegerOverflow=on
  state_cast7 : DataTypeConversion  OutDataTypeStr=fixdt(1, 46, 57)  SampleTime=1.62760416666667e-07  SaturateOnIntegerOverflow=on
  state_cast8 : DataTypeConversion  OutDataTypeStr=fixdt(1, 46, 44)  SampleTime=1.62760416666667e-07  SaturateOnIntegerOverflow=on
  state_cast9 : DataTypeConversion  OutDataTypeStr=fixdt(1, 46, 43)  SampleTime=1.62760416666667e-07  SaturateOnIntegerOverflow=on
  Vout : Outport
  wires:
  Vin/1 -> To Workspace1/1, Data Type Conversion/1
  Gvar1_N/1 -> Input_delay2/1, To Workspace15/1
  Gvar2_N/1 -> Input_delay3/1, To Workspace14/1
  Gvar3_N/1 -> Input_delay1/1, To Workspace13/1
  Gvar4_N/1 -> Input_delay4/1
  Comparator Logic/1(out_mod) -> Sum25/2, To Workspace2/1
  Comparator Logic/2(out_dem) -> Sum22/1, To Workspace6/1
  Data Type Conversion2/1 -> Input_delay5/1
  Delay Mod1/1 -> input_acc_cast14/1
  Delay Mod2/1 -> input_acc_cast6/1
  Delay Mod3/1 -> input_acc_cast8/1
  Delay Mod4/1 -> input_acc_cast9/1
  Delay Mod5/1 -> input_acc_cast7/1
  Delay Mod6/1 -> input_acc_cast12/1
  Delay Mod8/1 -> Z22_circuit/2(Z22_in)
  Delay Mod9/1 -> Z23_circuit/4(Data in)
  Delay1/1 -> input_acc_cast3/1
  Delay2/1 -> input_acc_cast1/1
  Delay3/1 -> Switch7/3, Relational Operator4/1
  Difference1/1(Y) -> Gain10/1
  Difference10/1(Y) -> Gain65/1
  Difference11/1(Y) -> Gain66/1
  Difference12/1(Y) -> Gain67/1
  Difference13/1(Y) -> Gain68/1
  Difference3/1(Y) -> Gain13/1
  Difference4/1(Y) -> Gain42/1
  Difference5/1(Y) -> Gain44/1
  Difference6/1(Y) -> Gain45/1
  Difference7/1(Y) -> Gain46/1
  Difference8/1(Y) -> Gain64/1
  Difference9/1(Y) -> Gain57/1
  Discrete-Time Integrator1_saturate/1 -> Discrete-Time Integrator1_reg/1, To Workspace12/1, Gain63/1, Gain62/1, Gain50/1
  Discrete-Time Integrator6_saturate/1 -> Discrete-Time Integrator6_reg/1, To Workspace8/1, To Workspace3/1, Gain59/1, Gain54/1, Gain53/1
  Gain20/1 -> Difference4/1(U)
  Gain27/1 -> Difference13/1(U)
  Gain28/1 -> Difference12/1(U)
  Gain29/1 -> Difference10/1(U)
  Gain30/1 -> Difference11/1(U)
  Gain33/1 -> Difference8/1(U)
  Gain34/1 -> Difference9/1(U)
  Gain54/1 -> Difference5/1(U)
  Gain56/1 -> Difference6/1(U)
  Gain59/1 -> Path Delay 4/1
  Gain62/1 -> Path Delay 5/1
  Gain63/1 -> Difference7/1(U)
  Gain9/1 -> Difference1/1(U)
  Input_delay1/1 -> "LUT_Gvar3 "/1, Z23_circuit/3(Gvar3_N), Z24_circuit/1(Gvar3_N)
  Input_delay2/1 -> "LUT_Gvar1 "/1, Z23_circuit/1(Gvar1_N), Z22_circuit/1(Gvar1_N)
  Input_delay3/1 -> LUT_Gvar2_rev/1, Z23_circuit/2(Gvar2_N), Z25_circuit/1(Gvar2_N)
  Input_delay4/1 -> 1-D Lookup Table1/1, To Workspace16/1
  "LUT_Gvar1 "/1 -> Mult_delay3/1
  LUT_Gvar2_rev/1 -> Mult_delay2/1
  "LUT_Gvar3 "/1 -> Mult_delay1/1
  Mult_delay1/1 -> Product3/1, Product2/1
  Mult_delay2/1 -> Product5/1, Product4/1
  Mult_delay3/1 -> Product/1, Product1/1
  Path Delay 0/1 -> input_acc_cast/1
  Path Delay 1/1 -> Difference3/1(U), To Workspace10/1, Gain5/1
  Path Delay 2/1 -> input_acc_cast15/1
  Path Delay 3/1 -> Comparator Logic/2(in_inverted)
  Path Delay 4/1 -> Sum21/2
  Path Delay 5/1 -> Sum14/2
  Product5/1 -> Z25_circuit/2(Z25_in)
  Rate Transition/1 -> Path Delay 0/1
  Rate Transition1/1 -> Data Type Conversion1/1
  Sum10/1 -> Delay2/1
  Sum11/1 -> Delay Mod8/1
  Sum13/1 -> Delay Mod9/1
  Sum15/1 -> Z24_circuit/2(Z24_in)
  Sum20/1 -> Delay Mod2/1
  Sum22/1 -> Delay Mod3/1
  Sum25/1 -> Delay Mod4/1
  Sum28/1 -> Delay Mod5/1
  Sum6/1 -> Delay Mod6/1
  Sum8/1 -> Delay Mod1/1
  Sum9/1 -> Delay1/1
  Switch4/1 -> Delay3/1
  Z22_circuit/1(Z22_out) -> Product1/2, Gain30/1
  Z23_circuit/1(Out1) -> Product3/2, Product/2, Product5/2, Gain34/1
  Z24_circuit/1(Z24_out) -> Product2/2, Gain27/1
  Z25_circuit/1(Z25_out) -> Product4/2
  Discrete-Time Integrator1_reg/1 -> adder1/1
  Discrete-Time Integrator2_reg/1 -> adder/1
  Discrete-Time Integrator4_reg/1 -> adder4/1
  Discrete-Time Integrator5_reg/1 -> adder3/1
  Discrete-Time Integrator6_reg/1 -> adder2/1
  state_cast/1 -> s_state_out1/1, nume_gain_b0/1
  s_state_out1/1 -> s_state_out2/1, nume_gain1/1, denom_gain1/1
  s_state_out2/1 -> s_state_out3/1, nume_gain2/1, denom_gain2/1
  s_state_out3/1 -> nume_gain3/1, denom_gain3/1
  state_cast15/1 -> s_state_out11/1, nume_gain_b015/1
  s_state_out11/1 -> nume_gain115/1, denom_gain115/1
  state_cast9/1 -> s_state_out12/1, nume_gain_b09/1
  s_state_out12/1 -> nume_gain19/1, denom_gain19/1
  state_cast8/1 -> s_state_out13/1, nume_gain_b08/1
  s_state_out13/1 -> nume_gain18/1, denom_gain18/1
  state_cast7/1 -> s_state_out14/1, nume_gain_b07/1
  s_state_out14/1 -> nume_gain15/1, denom_gain15/1
  state_cast14/1 -> s_state_out15/1, nume_gain_b014/1
  s_state_out15/1 -> nume_gain110/1, denom_gain110/1
  state_cast13/1 -> s_state_out16/1, nume_gain_b013/1
  s_state_out16/1 -> nume_gain111/1, denom_gain111/1
  state_cast10/1 -> s_state_out17/1, nume_gain_b010/1
  s_state_out17/1 -> nume_gain113/1, denom_gain113/1
  state_cast2/1 -> s_state_out18/1, nume_gain_b02/1
  s_state_out18/1 -> nume_gain12/1, denom_gain12/1
  state_cast1/1 -> s_state_out19/1, nume_gain_b01/1
  s_state_out19/1 -> nume_gain13/1, denom_gain13/1
  state_cast4/1 -> s_state_out110/1, nume_gain_b04/1
  s_state_out110/1 -> nume_gain14/1, denom_gain14/1
  state_cast6/1 -> s_state_out111/1, nume_gain_b06/1
  s_state_out111/1 -> nume_gain16/1, denom_gain16/1
  state_cast5/1 -> s_state_out112/1, nume_gain_b05/1
  s_state_out112/1 -> nume_gain17/1, denom_gain17/1
  state_cast3/1 -> s_state_out113/1, nume_gain_b03/1
  s_state_out113/1 -> nume_gain11/1, denom_gain11/1
  state_cast11/1 -> s_state_out114/1, nume_gain_b011/1
  s_state_out114/1 -> nume_gain114/1, denom_gain114/1
  state_cast12/1 -> s_state_out115/1, nume_gain_b012/1
  s_state_out115/1 -> nume_gain112/1, denom_gain112/1
  Input_delay5/1 -> Input_delay5_switch/1
  Input_delay5_ctrl_const/1 -> Input_delay5_ctrl_delay/1
  Input_delay5_ctrl_delay/1 -> Input_delay5_switch/2
  Compare To Zero2/1 -> Comparator Logic/3(clk_div)
  Constant8/1 -> Sum1/1
  Constant14/1 -> Switch7/1
  Gain5/1 -> Sum9/2
  Gain6/1 -> Sum5/1
  Discrete-Time Integrator2_saturate/1 -> Path Delay 2/1, Discrete-Time Integrator2_reg/1, To Workspace11/1, Gain9/1, Gain8/1
  Discrete-Time Integrator5_saturate/1 -> Discrete-Time Integrator5_reg/1, Comparator Logic/1(in_noninverted), To Workspace7/1, To Workspace5/1, Gain56/1, Gain55/1
  Discrete-Time Integrator4_saturate/1 -> Path Delay 3/1, Discrete-Time Integrator4_reg/1, To Workspace9/1, To Workspace4/1, Gain60/1, Gain20/1
  Data Type Conversion/1 -> Rate Transition/1
  input_acc_cast/1 -> denom_acc1/1
  denom_gain3/1 -> denom_acc_cast3/1
  denom_acc_cast3/1 -> denom_acc3/2
  denom_gain2/1 -> denom_acc_cast2/1
  denom_acc_cast2/1 -> denom_acc2/2
  denom_gain1/1 -> denom_acc_cast1/1
  denom_acc_cast1/1 -> denom_acc1/2
  denom_acc1/1 -> denom_acc2/1
  denom_acc2/1 -> denom_acc3/1
  denom_acc3/1 -> denom_scale_by_a0/1
  denom_scale_by_a0/1 -> state_cast/1
  nume_gain_b0/1 -> nume_gain_b0_cast/1
  nume_gain_b0_cast/1 -> s_nume_acc1/1
  nume_gain1/1 -> nume_acc_cast1/1
  nume_acc_cast1/1 -> s_nume_acc1/2
  s_nume_acc1/1 -> s_nume_acc2/1
  nume_gain2/1 -> nume_acc_cast2/1
  nume_acc_cast2/1 -> s_nume_acc2/2
  s_nume_acc2/1 -> s_nume_acc3/1
  nume_gain3/1 -> nume_acc_cast3/1
  nume_acc_cast3/1 -> s_nume_acc3/2
  s_nume_acc3/1 -> output_cast/1
  output_cast/1 -> Path Delay 1/1
  Gain13/1 -> Gain6/1
  1-D Lookup Table1/1 -> Data Type Conversion2/1
  Input_delay5_Initial_Val/1 -> Input_delay5_switch/3
  Input_delay5_switch/1 -> Relational Operator4/2, Relational Operator7/2
  Relational Operator7/1 -> Switch4/2
  Sum1/1 -> Switch4/1
  Relational Operator4/1 -> Switch7/2
  Switch7/1 -> Compare To Zero2/1, Switch4/3, Sum1/2, Relational Operator7/1
  nume_gain11/1 -> nume_acc_cast11/1
  nume_acc_cast11/1 -> s_nume_acc13/2
  denom_gain11/1 -> denom_acc_cast11/1
  denom_acc_cast11/1 -> denom_acc13/2
  nume_gain12/1 -> nume_acc_cast12/1
  nume_acc_cast12/1 -> s_nume_acc12/2
  denom_gain12/1 -> denom_acc_cast12/1
  denom_acc_cast12/1 -> denom_acc12/2
  nume_gain13/1 -> nume_acc_cast13/1
  nume_acc_cast13/1 -> s_nume_acc11/2
  denom_gain13/1 -> denom_acc_cast13/1
  denom_acc_cast13/1 -> denom_acc11/2
  Gain68/1 -> Sum10/2
  Gain25/1 -> Sum10/1
  input_acc_cast1/1 -> denom_acc11/1
  denom_acc11/1 -> denom_scale_by_a01/1
  denom_scale_by_a01/1 -> state_cast1/1
  nume_gain_b01/1 -> nume_gain_b0_cast1/1
  nume_gain_b0_cast1/1 -> s_nume_acc11/1
  s_nume_acc11/1 -> output_cast1/1
  output_cast1/1 -> s_output_cast_wire/1
  s_output_cast_wire/1 -> Gain28/1, Gain26/1
  Gain26/1 -> Sum3/2
  Gain23/1 -> Sum3/1
  Sum3/1 -> input_acc_cast2/1
  input_acc_cast2/1 -> denom_acc12/1
  denom_acc12/1 -> denom_scale_by_a02/1
  denom_scale_by_a02/1 -> state_cast2/1
  nume_gain_b02/1 -> nume_gain_b0_cast2/1
  nume_gain_b0_cast2/1 -> s_nume_acc12/1
  s_nume_acc12/1 -> output_cast2/1
  output_cast2/1 -> s_output_cast_wire1/1
  s_output_cast_wire1/1 -> Gain25/1, Gain24/1
  Gain24/1 -> Sum9/3
  Gain8/1 -> Sum2/2
  Gain10/1 -> Sum2/1
  Sum2/1 -> Sum9/1
  input_acc_cast3/1 -> denom_acc13/1
  denom_acc13/1 -> denom_scale_by_a03/1
  denom_scale_by_a03/1 -> state_cast3/1
  nume_gain_b03/1 -> nume_gain_b0_cast3/1
  nume_gain_b0_cast3/1 -> s_nume_acc13/1
  s_nume_acc13/1 -> output_cast3/1
  output_cast3/1 -> s_output_cast_wire2/1
  s_output_cast_wire2/1 -> Gain7/1, Gain23/1
  Gain7/1 -> dtc/1
  dtc/1 -> gain/1
  gain/1 -> dtc1/1
  dtc1/1 -> adder/2
  adder/1 -> Discrete-Time Integrator2_saturate/1
  nume_gain14/1 -> nume_acc_cast14/1
  nume_acc_cast14/1 -> s_nume_acc14/2
  denom_gain14/1 -> denom_acc_cast14/1
  denom_acc_cast14/1 -> denom_acc14/2
  Gain57/1 -> Sum14/1
  Sum14/1 -> input_acc_cast4/1
  input_acc_cast4/1 -> denom_acc14/1
  denom_acc14/1 -> denom_scale_by_a04/1
  denom_scale_by_a04/1 -> state_cast4/1
  nume_gain_b04/1 -> nume_gain_b0_cast4/1
  nume_gain_b0_cast4/1 -> s_nume_acc14/1
  s_nume_acc14/1 -> output_cast4/1
  output_cast4/1 -> s_output_cast_wire3/1
  s_output_cast_wire3/1 -> Gain33/1
  nume_gain15/1 -> nume_acc_cast15/1
  nume_acc_cast15/1 -> s_nume_acc17/2
  denom_gain15/1 -> denom_acc_cast15/1
  denom_acc_cast15/1 -> denom_acc17/2
  nume_gain16/1 -> nume_acc_cast16/1
  nume_acc_cast16/1 -> s_nume_acc16/2
  denom_gain16/1 -> denom_acc_cast16/1
  denom_acc_cast16/1 -> denom_acc16/2
  nume_gain17/1 -> nume_acc_cast17/1
  nume_acc_cast17/1 -> s_nume_acc15/2
  denom_gain17/1 -> denom_acc_cast17/1
  denom_acc_cast17/1 -> denom_acc15/2
  Gain48/1 -> Sum21/1
  Sum21/1 -> input_acc_cast5/1
  input_acc_cast5/1 -> denom_acc15/1
  denom_acc15/1 -> denom_scale_by_a05/1
  denom_scale_by_a05/1 -> state_cast5/1
  nume_gain_b05/1 -> nume_gain_b0_cast5/1
  nume_gain_b0_cast5/1 -> s_nume_acc15/1
  s_nume_acc15/1 -> output_cast5/1
  output_cast5/1 -> s_output_cast_wire4/1
  s_output_cast_wire4/1 -> Gain47/1
  Gain47/1 -> Sum20/3
  Gain50/1 -> Sum20/2
  Gain49/1 -> Sum20/1
  input_acc_cast6/1 -> denom_acc16/1
  denom_acc16/1 -> denom_scale_by_a06/1
  denom_scale_by_a06/1 -> state_cast6/1
  nume_gain_b06/1 -> nume_gain_b0_cast6/1
  nume_gain_b0_cast6/1 -> s_nume_acc16/1
  s_nume_acc16/1 -> output_cast6/1
  output_cast6/1 -> s_output_cast_wire5/1
  s_output_cast_wire5/1 -> Gain48/1, Gain43/1
  Gain43/1 -> Sum28/2
  Gain46/1 -> Sum28/1
  input_acc_cast7/1 -> denom_acc17/1
  denom_acc17/1 -> denom_scale_by_a07/1
  denom_scale_by_a07/1 -> state_cast7/1
  nume_gain_b07/1 -> nume_gain_b0_cast7/1
  nume_gain_b0_cast7/1 -> s_nume_acc17/1
  s_nume_acc17/1 -> output_cast7/1
  output_cast7/1 -> s_output_cast_wire6/1
  s_output_cast_wire6/1 -> Gain61/1, Gain49/1
  Gain61/1 -> dtc2/1
  dtc2/1 -> gain1/1
  gain1/1 -> dtc3/1
  dtc3/1 -> adder1/2
  adder1/1 -> Discrete-Time Integrator1_saturate/1
  nume_gain18/1 -> nume_acc_cast18/1
  nume_acc_cast18/1 -> s_nume_acc18/2
  denom_gain18/1 -> denom_acc_cast18/1
  denom_acc_cast18/1 -> denom_acc18/2
  Gain44/1 -> Sum23/2
  Gain53/1 -> Sum23/1
  Sum23/1 -> Sum22/2
  input_acc_cast8/1 -> denom_acc18/1
  denom_acc18/1 -> denom_scale_by_a08/1
  denom_scale_by_a08/1 -> state_cast8/1
  nume_gain_b08/1 -> nume_gain_b0_cast8/1
  nume_gain_b0_cast8/1 -> s_nume_acc18/1
  s_nume_acc18/1 -> output_cast8/1
  output_cast8/1 -> s_output_cast_wire7/1
  s_output_cast_wire7/1 -> Gain52/1
  Gain52/1 -> dtc4/1
  dtc4/1 -> gain2/1
  gain2/1 -> dtc5/1
  dtc5/1 -> adder2/2
  adder2/1 -> Discrete-Time Integrator6_saturate/1
  nume_gain19/1 -> nume_acc_cast19/1
  nume_acc_cast19/1 -> s_nume_acc19/2
  denom_gain19/1 -> denom_acc_cast19/1
  denom_acc_cast19/1 -> denom_acc19/2
  Gain55/1 -> Sum24/2
  Gain45/1 -> Sum24/1
  Sum24/1 -> Sum25/1
  input_acc_cast9/1 -> denom_acc19/1
  denom_acc19/1 -> denom_scale_by_a09/1
  denom_scale_by_a09/1 -> state_cast9/1
  nume_gain_b09/1 -> nume_gain_b0_cast9/1
  nume_gain_b0_cast9/1 -> s_nume_acc19/1
  s_nume_acc19/1 -> output_cast9/1
  output_cast9/1 -> s_output_cast_wire8/1
  s_output_cast_wire8/1 -> Gain51/1
  Gain51/1 -> dtc6/1
  dtc6/1 -> gain3/1
  gain3/1 -> dtc7/1
  dtc7/1 -> adder3/2
  adder3/1 -> Discrete-Time Integrator5_saturate/1
  Gain64/1 -> Sum13/3
  Product1/1 -> Sum13/2
  Product4/1 -> Sum18/2
  Product2/1 -> Sum18/1
  Sum18/1 -> Sum13/1
  nume_gain110/1 -> nume_acc_cast110/1
  nume_acc_cast110/1 -> s_nume_acc114/2
  denom_gain110/1 -> denom_acc_cast110/1
  denom_acc_cast110/1 -> denom_acc114/2
  Gain42/1 -> Sum8/2
  nume_gain111/1 -> nume_acc_cast111/1
  nume_acc_cast111/1 -> s_nume_acc113/2
  denom_gain111/1 -> denom_acc_cast111/1
  denom_acc_cast111/1 -> denom_acc113/2
  Gain17/1 -> Sum7/3
  Gain60/1 -> Sum7/2
  nume_gain112/1 -> nume_acc_cast112/1
  nume_acc_cast112/1 -> s_nume_acc112/2
  denom_gain112/1 -> denom_acc_cast112/1
  denom_acc_cast112/1 -> denom_acc112/2
  Gain15/1 -> Sum6/3
  nume_gain113/1 -> nume_acc_cast113/1
  nume_acc_cast113/1 -> s_nume_acc110/2
  denom_gain113/1 -> denom_acc_cast113/1
  denom_acc_cast113/1 -> denom_acc110/2
  Gain66/1 -> Sum12/2
  Gain32/1 -> Sum12/1
  Sum12/1 -> input_acc_cast10/1
  input_acc_cast10/1 -> denom_acc110/1
  denom_acc110/1 -> denom_scale_by_a010/1
  denom_scale_by_a010/1 -> state_cast10/1
  nume_gain_b010/1 -> nume_gain_b0_cast10/1
  nume_gain_b0_cast10/1 -> s_nume_acc110/1
  s_nume_acc110/1 -> output_cast10/1
  output_cast10/1 -> s_output_cast_wire9/1
  s_output_cast_wire9/1 -> Gain31/1, Gain29/1
  Gain31/1 -> Sum6/2
  nume_gain114/1 -> nume_acc_cast114/1
  nume_acc_cast114/1 -> s_nume_acc111/2
  denom_gain114/1 -> denom_acc_cast114/1
  denom_acc_cast114/1 -> denom_acc111/2
  Gain14/1 -> Sum5/2
  Sum5/1 -> input_acc_cast11/1
  input_acc_cast11/1 -> denom_acc111/1
  denom_acc111/1 -> denom_scale_by_a011/1
  denom_scale_by_a011/1 -> state_cast11/1
  nume_gain_b011/1 -> nume_gain_b0_cast11/1
  nume_gain_b0_cast11/1 -> s_nume_acc111/1
  s_nume_acc111/1 -> output_cast11/1
  output_cast11/1 -> s_output_cast_wire10/1
  s_output_cast_wire10/1 -> Gain12/1
  Gain12/1 -> Sum6/1
  input_acc_cast12/1 -> denom_acc112/1
  denom_acc112/1 -> denom_scale_by_a012/1
  denom_scale_by_a012/1 -> state_cast12/1
  nume_gain_b012/1 -> nume_gain_b0_cast12/1
  nume_gain_b0_cast12/1 -> s_nume_acc112/1
  s_nume_acc112/1 -> output_cast12/1
  output_cast12/1 -> s_output_cast_wire11/1
  s_output_cast_wire11/1 -> Gain32/1, Gain16/1, Gain14/1
  Gain16/1 -> Sum7/1
  Sum7/1 -> input_acc_cast13/1
  input_acc_cast13/1 -> denom_acc113/1
  denom_acc113/1 -> denom_scale_by_a013/1
  denom_scale_by_a013/1 -> state_cast13/1
  nume_gain_b013/1 -> nume_gain_b0_cast13/1
  nume_gain_b0_cast13/1 -> s_nume_acc113/1
  s_nume_acc113/1 -> output_cast13/1
  output_cast13/1 -> s_output_cast_wire12/1
  s_output_cast_wire12/1 -> Gain18/1, Gain15/1
  Gain18/1 -> Sum8/1
  input_acc_cast14/1 -> denom_acc114/1
  denom_acc114/1 -> denom_scale_by_a014/1
  denom_scale_by_a014/1 -> state_cast14/1
  nume_gain_b014/1 -> nume_gain_b0_cast14/1
  nume_gain_b0_cast14/1 -> s_nume_acc114/1
  s_nume_acc114/1 -> output_cast14/1
  output_cast14/1 -> s_output_cast_wire13/1
  s_output_cast_wire13/1 -> Gain19/1, Gain17/1
  Gain19/1 -> dtc8/1
  dtc8/1 -> gain4/1
  gain4/1 -> dtc9/1
  dtc9/1 -> adder4/2
  adder4/1 -> Discrete-Time Integrator4_saturate/1
  Product/1 -> Sum11/2
  Gain65/1 -> Sum11/1
  Product3/1 -> Sum15/2
  Gain67/1 -> Sum15/1
  input_acc_cast15/1 -> denom_acc115/1
  denom_gain115/1 -> denom_acc_cast115/1
  denom_acc_cast115/1 -> denom_acc115/2
  denom_acc115/1 -> denom_scale_by_a015/1
  denom_scale_by_a015/1 -> state_cast15/1
  nume_gain_b015/1 -> s_nume_acc115/1
  nume_gain115/1 -> s_nume_acc115/2
  s_nume_acc115/1 -> output_cast15/1
  output_cast15/1 -> Rate Transition1/1
  Data Type Conversion1/1 -> Vout/1
